simulink model "model"  (R2014a)
(part 2 of 3)

  _CN_86577898_150000_CN_136543640_150000 : powerlib/Elements/Distributed Parameters Line  Phases=3  Frequency=60  Resistance=[0.01273 0.3864]  Inductance="[0.9337e-3  4.1264e-3]"  Capacitance=[12.74e-9 7.751e-9]  Length=52.261  x1=[0 0 0 0; 0.0001244 0 0 0; 0.0002488 0 0 0; 0.0003733 0 0 0; 0.0004977 0 0 0; 0.0006221 0 0 0]  x2=[0 0 0 0; 0.0001244 0 0 0; 0.0002488 0 0 0; 0.0003733 0 0 0; 0.0004977 0 0 0; 0.0006221 0 0 0]  x3=[0 0 0 0; 0.0001244 0 0 0; 0.0002488 0 0 0; 0.0003733 0 0 0; 0.0004977 0 0 0; 0.0006221 0 0 0]  x4=[0 0 0 0; 0.0001244 0 0 0; 0.0002488 0 0 0; 0.0003733 0 0 0; 0.0004977 0 0 0; 0.0006221 0 0 0]  x5=0  V1=ones(3,3)  V2=ones(3,3)  I1=ones(3,3)  I2=ones(3,3)  nHarmo=1  Measurements=None
  _CN_92352843_150000_CN_149922043_150000 : powerlib/Elements/Distributed Parameters Line  Phases=3  Frequency=60  Resistance=[0.01273 0.3864]  Inductance="[0.9337e-3  4.1264e-3]"  Capacitance=[12.74e-9 7.751e-9]  Length=68.3675  x1=[0 0 0 0; 0.0001244 0 0 0; 0.0002488 0 0 0; 0.0003733 0 0 0; 0.0004977 0 0 0; 0.0006221 0 0 0]  x2=[0 0 0 0; 0.0001244 0 0 0; 0.0002488 0 0 0; 0.0003733 0 0 0; 0.0004977 0 0 0; 0.0006221 0 0 0]  x3=[0 0 0 0; 0.0001244 0 0 0; 0.0002488 0 0 0; 0.0003733 0 0 0; 0.0004977 0 0 0; 0.0006221 0 0 0]  x4=[0 0 0 0; 0.0001244 0 0 0; 0.0002488 0 0 0; 0.0003733 0 0 0; 0.0004977 0 0 0; 0.0006221 0 0 0]  x5=0  V1=ones(3,3)  V2=ones(3,3)  I1=ones(3,3)  I2=ones(3,3)  nHarmo=1  Measurements=None
  _CN_92611147_150000_CN_85646787_150000 : powerlib/Elements/Distributed Parameters Line  Phases=3  Frequency=60  Resistance=[0.01273 0.3864]  Inductance="[0.9337e-3  4.1264e-3]"  Capacitance=[12.74e-9 7.751e-9]  Length=4.1516  x1=[0 0 0 0; 0.0001244 0 0 0; 0.0002488 0 0 0; 0.0003733 0 0 0; 0.0004977 0 0 0; 0.0006221 0 0 0]  x2=[0 0 0 0; 0.0001244 0 0 0; 0.0002488 0 0 0; 0.0003733 0 0 0; 0.0004977 0 0 0; 0.0006221 0 0 0]  x3=[0 0 0 0; 0.0001244 0 0 0; 0.0002488 0 0 0; 0.0003733 0 0 0; 0.0004977 0 0 0; 0.0006221 0 0 0]  x4=[0 0 0 0; 0.0001244 0 0 0; 0.0002488 0 0 0; 0.0003733 0 0 0; 0.0004977 0 0 0; 0.0006221 0 0 0]  x5=0  V1=ones(3,3)  V2=ones(3,3)  I1=ones(3,3)  I2=ones(3,3)  nHarmo=1  Measurements=None
  _CN_92611161_150000_CN_85646787_150000 : powerlib/Elements/Distributed Parameters Line  Phases=3  Frequency=60  Resistance=[0.01273 0.3864]  Inductance="[0.9337e-3  4.1264e-3]"  Capacitance=[12.74e-9 7.751e-9]  Length=18.2958  x1=[0 0 0 0; 0.0001244 0 0 0; 0.0002488 0 0 0; 0.0003733 0 0 0; 0.0004977 0 0 0; 0.0006221 0 0 0]  x2=[0 0 0 0; 0.0001244 0 0 0; 0.0002488 0 0 0; 0.0003733 0 0 0; 0.0004977 0 0 0; 0.0006221 0 0 0]  x3=[0 0 0 0; 0.0001244 0 0 0; 0.0002488 0 0 0; 0.0003733 0 0 0; 0.0004977 0 0 0; 0.0006221 0 0 0]  x4=[0 0 0 0; 0.0001244 0 0 0; 0.0002488 0 0 0; 0.0003733 0 0 0; 0.0004977 0 0 0; 0.0006221 0 0 0]  x5=0  V1=ones(3,3)  V2=ones(3,3)  I1=ones(3,3)  I2=ones(3,3)  nHarmo=1  Measurements=None
  _CN_92611161_150000_CN_92611154_150000 : powerlib/Elements/Distributed Parameters Line  Phases=3  Frequency=60  Resistance=[0.01273 0.3864]  Inductance="[0.9337e-3  4.1264e-3]"  Capacitance=[12.74e-9 7.751e-9]  Length=4.6182  x1=[0 0 0 0; 0.0001244 0 0 0; 0.0002488 0 0 0; 0.0003733 0 0 0; 0.0004977 0 0 0; 0.0006221 0 0 0]  x2=[0 0 0 0; 0.0001244 0 0 0; 0.0002488 0 0 0; 0.0003733 0 0 0; 0.0004977 0 0 0; 0.0006221 0 0 0]  x3=[0 0 0 0; 0.0001244 0 0 0; 0.0002488 0 0 0; 0.0003733 0 0 0; 0.0004977 0 0 0; 0.0006221 0 0 0]  x4=[0 0 0 0; 0.0001244 0 0 0; 0.0002488 0 0 0; 0.0003733 0 0 0; 0.0004977 0 0 0; 0.0006221 0 0 0]  x5=0  V1=ones(3,3)  V2=ones(3,3)  I1=ones(3,3)  I2=ones(3,3)  nHarmo=1  Measurements=None
  _CN_93061385_150000_CN_93061390_150000 : powerlib/Elements/Distributed Parameters Line  Phases=3  Frequency=60  Resistance=[0.01273 0.3864]  Inductance="[0.9337e-3  4.1264e-3]"  Capacitance=[12.74e-9 7.751e-9]  Length=5.508  x1=[0 0 0 0; 0.0001244 0 0 0; 0.0002488 0 0 0; 0.0003733 0 0 0; 0.0004977 0 0 0; 0.0006221 0 0 0]  x2=[0 0 0 0; 0.0001244 0 0 0; 0.0002488 0 0 0; 0.0003733 0 0 0; 0.0004977 0 0 0; 0.0006221 0 0 0]  x3=[0 0 0 0; 0.0001244 0 0 0; 0.0002488 0 0 0; 0.0003733 0 0 0; 0.0004977 0 0 0; 0.0006221 0 0 0]  x4=[0 0 0 0; 0.0001244 0 0 0; 0.0002488 0 0 0; 0.0003733 0 0 0; 0.0004977 0 0 0; 0.0006221 0 0 0]  x5=0  V1=ones(3,3)  V2=ones(3,3)  I1=ones(3,3)  I2=ones(3,3)  nHarmo=1  Measurements=None
  _CN_93061390_150000_CN_115027244_150000 : powerlib/Elements/Distributed Parameters Line  Phases=3  Frequency=60  Resistance=[0.01273 0.3864]  Inductance="[0.9337e-3  4.1264e-3]"  Capacitance=[12.74e-9 7.751e-9]  Length=7.1152  x1=[0 0 0 0; 0.0001244 0 0 0; 0.0002488 0 0 0; 0.0003733 0 0 0; 0.0004977 0 0 0; 0.0006221 0 0 0]  x2=[0 0 0 0; 0.0001244 0 0 0; 0.0002488 0 0 0; 0.0003733 0 0 0; 0.0004977 0 0 0; 0.0006221 0 0 0]  x3=[0 0 0 0; 0.0001244 0 0 0; 0.0002488 0 0 0; 0.0003733 0 0 0; 0.0004977 0 0 0; 0.0006221 0 0 0]  x4=[0 0 0 0; 0.0001244 0 0 0; 0.0002488 0 0 0; 0.0003733 0 0 0; 0.0004977 0 0 0; 0.0006221 0 0 0]  x5=0  V1=ones(3,3)  V2=ones(3,3)  I1=ones(3,3)  I2=ones(3,3)  nHarmo=1  Measurements=None
  _CN_93085785_150000_CN_93085804_150000 : powerlib/Elements/Distributed Parameters Line  Phases=3  Frequency=60  Resistance=[0.01273 0.3864]  Inductance="[0.9337e-3  4.1264e-3]"  Capacitance=[12.74e-9 7.751e-9]  Length=0.70246  x1=[0 0 0 0; 0.0001244 0 0 0; 0.0002488 0 0 0; 0.0003733 0 0 0; 0.0004977 0 0 0; 0.0006221 0 0 0]  x2=[0 0 0 0; 0.0001244 0 0 0; 0.0002488 0 0 0; 0.0003733 0 0 0; 0.0004977 0 0 0; 0.0006221 0 0 0]  x3=[0 0 0 0; 0.0001244 0 0 0; 0.0002488 0 0 0; 0.0003733 0 0 0; 0.0004977 0 0 0; 0.0006221 0 0 0]  x4=[0 0 0 0; 0.0001244 0 0 0; 0.0002488 0 0 0; 0.0003733 0 0 0; 0.0004977 0 0 0; 0.0006221 0 0 0]  x5=0  V1=ones(3,3)  V2=ones(3,3)  I1=ones(3,3)  I2=ones(3,3)  nHarmo=1  Measurements=None
  _CN_93085804_150000_CN_93061390_150000 : powerlib/Elements/Distributed Parameters Line  Phases=3  Frequency=60  Resistance=[0.01273 0.3864]  Inductance="[0.9337e-3  4.1264e-3]"  Capacitance=[12.74e-9 7.751e-9]  Length=9.0251  x1=[0 0 0 0; 0.0001244 0 0 0; 0.0002488 0 0 0; 0.0003733 0 0 0; 0.0004977 0 0 0; 0.0006221 0 0 0]  x2=[0 0 0 0; 0.0001244 0 0 0; 0.0002488 0 0 0; 0.0003733 0 0 0; 0.0004977 0 0 0; 0.0006221 0 0 0]  x3=[0 0 0 0; 0.0001244 0 0 0; 0.0002488 0 0 0; 0.0003733 0 0 0; 0.0004977 0 0 0; 0.0006221 0 0 0]  x4=[0 0 0 0; 0.0001244 0 0 0; 0.0002488 0 0 0; 0.0003733 0 0 0; 0.0004977 0 0 0; 0.0006221 0 0 0]  x5=0  V1=ones(3,3)  V2=ones(3,3)  I1=ones(3,3)  I2=ones(3,3)  nHarmo=1  Measurements=None
  _CN_93119207_400000_CN_86577898_400000 : powerlib/Elements/Distributed Parameters Line  Phases=3  Frequency=60  Resistance=[0.01273 0.3864]  Inductance="[0.9337e-3  4.1264e-3]"  Capacitance=[12.74e-9 7.751e-9]  Length=76.386  x1=[0 0 0 0; 0.0001244 0 0 0; 0.0002488 0 0 0; 0.0003733 0 0 0; 0.0004977 0 0 0; 0.0006221 0 0 0]  x2=[0 0 0 0; 0.0001244 0 0 0; 0.0002488 0 0 0; 0.0003733 0 0 0; 0.0004977 0 0 0; 0.0006221 0 0 0]  x3=[0 0 0 0; 0.0001244 0 0 0; 0.0002488 0 0 0; 0.0003733 0 0 0; 0.0004977 0 0 0; 0.0006221 0 0 0]  x4=[0 0 0 0; 0.0001244 0 0 0; 0.0002488 0 0 0; 0.0003733 0 0 0; 0.0004977 0 0 0; 0.0006221 0 0 0]  x5=0  V1=ones(3,3)  V2=ones(3,3)  I1=ones(3,3)  I2=ones(3,3)  nHarmo=1  Measurements=None
  _CN_93173562_150000_CN_93172457_150000 : powerlib/Elements/Distributed Parameters Line  Phases=3  Frequency=60  Resistance=[0.01273 0.3864]  Inductance="[0.9337e-3  4.1264e-3]"  Capacitance=[12.74e-9 7.751e-9]  Length=18.3315  x1=[0 0 0 0; 0.0001244 0 0 0; 0.0002488 0 0 0; 0.0003733 0 0 0; 0.0004977 0 0 0; 0.0006221 0 0 0]  x2=[0 0 0 0; 0.0001244 0 0 0; 0.0002488 0 0 0; 0.0003733 0 0 0; 0.0004977 0 0 0; 0.0006221 0 0 0]  x3=[0 0 0 0; 0.0001244 0 0 0; 0.0002488 0 0 0; 0.0003733 0 0 0; 0.0004977 0 0 0; 0.0006221 0 0 0]  x4=[0 0 0 0; 0.0001244 0 0 0; 0.0002488 0 0 0; 0.0003733 0 0 0; 0.0004977 0 0 0; 0.0006221 0 0 0]  x5=0  V1=ones(3,3)  V2=ones(3,3)  I1=ones(3,3)  I2=ones(3,3)  nHarmo=1  Measurements=None
  _CN_93383685_150000_CN_135706289_150000 : powerlib/Elements/Distributed Parameters Line  Phases=3  Frequency=60  Resistance=[0.01273 0.3864]  Inductance="[0.9337e-3  4.1264e-3]"  Capacitance=[12.74e-9 7.751e-9]  Length=36.1686  x1=[0 0 0 0; 0.0001244 0 0 0; 0.0002488 0 0 0; 0.0003733 0 0 0; 0.0004977 0 0 0; 0.0006221 0 0 0]  x2=[0 0 0 0; 0.0001244 0 0 0; 0.0002488 0 0 0; 0.0003733 0 0 0; 0.0004977 0 0 0; 0.0006221 0 0 0]  x3=[0 0 0 0; 0.0001244 0 0 0; 0.0002488 0 0 0; 0.0003733 0 0 0; 0.0004977 0 0 0; 0.0006221 0 0 0]  x4=[0 0 0 0; 0.0001244 0 0 0; 0.0002488 0 0 0; 0.0003733 0 0 0; 0.0004977 0 0 0; 0.0006221 0 0 0]  x5=0  V1=ones(3,3)  V2=ones(3,3)  I1=ones(3,3)  I2=ones(3,3)  nHarmo=1  Measurements=None
  _CN_93383685_150000_CN_15642023_150000 : powerlib/Elements/Distributed Parameters Line  Phases=3  Frequency=60  Resistance=[0.01273 0.3864]  Inductance="[0.9337e-3  4.1264e-3]"  Capacitance=[12.74e-9 7.751e-9]  Length=0.77584  x1=[0 0 0 0; 0.0001244 0 0 0; 0.0002488 0 0 0; 0.0003733 0 0 0; 0.0004977 0 0 0; 0.0006221 0 0 0]  x2=[0 0 0 0; 0.0001244 0 0 0; 0.0002488 0 0 0; 0.0003733 0 0 0; 0.0004977 0 0 0; 0.0006221 0 0 0]  x3=[0 0 0 0; 0.0001244 0 0 0; 0.0002488 0 0 0; 0.0003733 0 0 0; 0.0004977 0 0 0; 0.0006221 0 0 0]  x4=[0 0 0 0; 0.0001244 0 0 0; 0.0002488 0 0 0; 0.0003733 0 0 0; 0.0004977 0 0 0; 0.0006221 0 0 0]  x5=0  V1=ones(3,3)  V2=ones(3,3)  I1=ones(3,3)  I2=ones(3,3)  nHarmo=1  Measurements=None
  _CN_93383685_400000_CN_149672244_400000 : powerlib/Elements/Distributed Parameters Line  Phases=3  Frequency=60  Resistance=[0.01273 0.3864]  Inductance="[0.9337e-3  4.1264e-3]"  Capacitance=[12.74e-9 7.751e-9]  Length=35.3897  x1=[0 0 0 0; 0.0001244 0 0 0; 0.0002488 0 0 0; 0.0003733 0 0 0; 0.0004977 0 0 0; 0.0006221 0 0 0]  x2=[0 0 0 0; 0.0001244 0 0 0; 0.0002488 0 0 0; 0.0003733 0 0 0; 0.0004977 0 0 0; 0.0006221 0 0 0]  x3=[0 0 0 0; 0.0001244 0 0 0; 0.0002488 0 0 0; 0.0003733 0 0 0; 0.0004977 0 0 0; 0.0006221 0 0 0]  x4=[0 0 0 0; 0.0001244 0 0 0; 0.0002488 0 0 0; 0.0003733 0 0 0; 0.0004977 0 0 0; 0.0006221 0 0 0]  x5=0  V1=ones(3,3)  V2=ones(3,3)  I1=ones(3,3)  I2=ones(3,3)  nHarmo=1  Measurements=None
  _CN_93383685_400000_CN_15641949_400000 : powerlib/Elements/Distributed Parameters Line  Phases=3  Frequency=60  Resistance=[0.01273 0.3864]  Inductance="[0.9337e-3  4.1264e-3]"  Capacitance=[12.74e-9 7.751e-9]  Length=15.3876  x1=[0 0 0 0; 0.0001244 0 0 0; 0.0002488 0 0 0; 0.0003733 0 0 0; 0.0004977 0 0 0; 0.0006221 0 0 0]  x2=[0 0 0 0; 0.0001244 0 0 0; 0.0002488 0 0 0; 0.0003733 0 0 0; 0.0004977 0 0 0; 0.0006221 0 0 0]  x3=[0 0 0 0; 0.0001244 0 0 0; 0.0002488 0 0 0; 0.0003733 0 0 0; 0.0004977 0 0 0; 0.0006221 0 0 0]  x4=[0 0 0 0; 0.0001244 0 0 0; 0.0002488 0 0 0; 0.0003733 0 0 0; 0.0004977 0 0 0; 0.0006221 0 0 0]  x5=0  V1=ones(3,3)  V2=ones(3,3)  I1=ones(3,3)  I2=ones(3,3)  nHarmo=1  Measurements=None
  _CN_93383685_400000_CN_15642023_150000 : powerlib/Elements/Distributed Parameters Line  Phases=3  Frequency=60  Resistance=[0.01273 0.3864]  Inductance="[0.9337e-3  4.1264e-3]"  Capacitance=[12.74e-9 7.751e-9]  Length=0.4473  x1=[0 0 0 0; 0.0001244 0 0 0; 0.0002488 0 0 0; 0.0003733 0 0 0; 0.0004977 0 0 0; 0.0006221 0 0 0]  x2=[0 0 0 0; 0.0001244 0 0 0; 0.0002488 0 0 0; 0.0003733 0 0 0; 0.0004977 0 0 0; 0.0006221 0 0 0]  x3=[0 0 0 0; 0.0001244 0 0 0; 0.0002488 0 0 0; 0.0003733 0 0 0; 0.0004977 0 0 0; 0.0006221 0 0 0]  x4=[0 0 0 0; 0.0001244 0 0 0; 0.0002488 0 0 0; 0.0003733 0 0 0; 0.0004977 0 0 0; 0.0006221 0 0 0]  x5=0  V1=ones(3,3)  V2=ones(3,3)  I1=ones(3,3)  I2=ones(3,3)  nHarmo=1  Measurements=None
  _CN_93383685_400000_CN_171506480_400000 : powerlib/Elements/Distributed Parameters Line  Phases=3  Frequency=60  Resistance=[0.01273 0.3864]  Inductance="[0.9337e-3  4.1264e-3]"  Capacitance=[12.74e-9 7.751e-9]  Length=49.411  x1=[0 0 0 0; 0.0001244 0 0 0; 0.0002488 0 0 0; 0.0003733 0 0 0; 0.0004977 0 0 0; 0.0006221 0 0 0]  x2=[0 0 0 0; 0.0001244 0 0 0; 0.0002488 0 0 0; 0.0003733 0 0 0; 0.0004977 0 0 0; 0.0006221 0 0 0]  x3=[0 0 0 0; 0.0001244 0 0 0; 0.0002488 0 0 0; 0.0003733 0 0 0; 0.0004977 0 0 0; 0.0006221 0 0 0]  x4=[0 0 0 0; 0.0001244 0 0 0; 0.0002488 0 0 0; 0.0003733 0 0 0; 0.0004977 0 0 0; 0.0006221 0 0 0]  x5=0  V1=ones(3,3)  V2=ones(3,3)  I1=ones(3,3)  I2=ones(3,3)  nHarmo=1  Measurements=None
  _CN_93383685_400000_CN_249066440_400000 : powerlib/Elements/Distributed Parameters Line  Phases=3  Frequency=60  Resistance=[0.01273 0.3864]  Inductance="[0.9337e-3  4.1264e-3]"  Capacitance=[12.74e-9 7.751e-9]  Length=18.7994  x1=[0 0 0 0; 0.0001244 0 0 0; 0.0002488 0 0 0; 0.0003733 0 0 0; 0.0004977 0 0 0; 0.0006221 0 0 0]  x2=[0 0 0 0; 0.0001244 0 0 0; 0.0002488 0 0 0; 0.0003733 0 0 0; 0.0004977 0 0 0; 0.0006221 0 0 0]  x3=[0 0 0 0; 0.0001244 0 0 0; 0.0002488 0 0 0; 0.0003733 0 0 0; 0.0004977 0 0 0; 0.0006221 0 0 0]  x4=[0 0 0 0; 0.0001244 0 0 0; 0.0002488 0 0 0; 0.0003733 0 0 0; 0.0004977 0 0 0; 0.0006221 0 0 0]  x5=0  V1=ones(3,3)  V2=ones(3,3)  I1=ones(3,3)  I2=ones(3,3)  nHarmo=1  Measurements=None
  _CN_93383685_400000_CN_86577898_400000 : powerlib/Elements/Distributed Parameters Line  Phases=3  Frequency=60  Resistance=[0.01273 0.3864]  Inductance="[0.9337e-3  4.1264e-3]"  Capacitance=[12.74e-9 7.751e-9]  Length=53.9293  x1=[0 0 0 0; 0.0001244 0 0 0; 0.0002488 0 0 0; 0.0003733 0 0 0; 0.0004977 0 0 0; 0.0006221 0 0 0]  x2=[0 0 0 0; 0.0001244 0 0 0; 0.0002488 0 0 0; 0.0003733 0 0 0; 0.0004977 0 0 0; 0.0006221 0 0 0]  x3=[0 0 0 0; 0.0001244 0 0 0; 0.0002488 0 0 0; 0.0003733 0 0 0; 0.0004977 0 0 0; 0.0006221 0 0 0]  x4=[0 0 0 0; 0.0001244 0 0 0; 0.0002488 0 0 0; 0.0003733 0 0 0; 0.0004977 0 0 0; 0.0006221 0 0 0]  x5=0  V1=ones(3,3)  V2=ones(3,3)  I1=ones(3,3)  I2=ones(3,3)  nHarmo=1  Measurements=None
  _CN_93906290_150000_CN_93906327_150000 : powerlib/Elements/Distributed Parameters Line  Phases=3  Frequency=60  Resistance=[0.01273 0.3864]  Inductance="[0.9337e-3  4.1264e-3]"  Capacitance=[12.74e-9 7.751e-9]  Length=20.4524  x1=[0 0 0 0; 0.0001244 0 0 0; 0.0002488 0 0 0; 0.0003733 0 0 0; 0.0004977 0 0 0; 0.0006221 0 0 0]  x2=[0 0 0 0; 0.0001244 0 0 0; 0.0002488 0 0 0; 0.0003733 0 0 0; 0.0004977 0 0 0; 0.0006221 0 0 0]  x3=[0 0 0 0; 0.0001244 0 0 0; 0.0002488 0 0 0; 0.0003733 0 0 0; 0.0004977 0 0 0; 0.0006221 0 0 0]  x4=[0 0 0 0; 0.0001244 0 0 0; 0.0002488 0 0 0; 0.0003733 0 0 0; 0.0004977 0 0 0; 0.0006221 0 0 0]  x5=0  V1=ones(3,3)  V2=ones(3,3)  I1=ones(3,3)  I2=ones(3,3)  nHarmo=1  Measurements=None
  _CN_95989793_150000_CN_92352843_150000 : powerlib/Elements/Distributed Parameters Line  Phases=3  Frequency=60  Resistance=[0.01273 0.3864]  Inductance="[0.9337e-3  4.1264e-3]"  Capacitance=[12.74e-9 7.751e-9]  Length=5.9887  x1=[0 0 0 0; 0.0001244 0 0 0; 0.0002488 0 0 0; 0.0003733 0 0 0; 0.0004977 0 0 0; 0.0006221 0 0 0]  x2=[0 0 0 0; 0.0001244 0 0 0; 0.0002488 0 0 0; 0.0003733 0 0 0; 0.0004977 0 0 0; 0.0006221 0 0 0]  x3=[0 0 0 0; 0.0001244 0 0 0; 0.0002488 0 0 0; 0.0003733 0 0 0; 0.0004977 0 0 0; 0.0006221 0 0 0]  x4=[0 0 0 0; 0.0001244 0 0 0; 0.0002488 0 0 0; 0.0003733 0 0 0; 0.0004977 0 0 0; 0.0006221 0 0 0]  x5=0  V1=ones(3,3)  V2=ones(3,3)  I1=ones(3,3)  I2=ones(3,3)  nHarmo=1  Measurements=None
  _CN_96020492_150000_CN_96314289_150000 : powerlib/Elements/Distributed Parameters Line  Phases=3  Frequency=60  Resistance=[0.01273 0.3864]  Inductance="[0.9337e-3  4.1264e-3]"  Capacitance=[12.74e-9 7.751e-9]  Length=14.9727  x1=[0 0 0 0; 0.0001244 0 0 0; 0.0002488 0 0 0; 0.0003733 0 0 0; 0.0004977 0 0 0; 0.0006221 0 0 0]  x2=[0 0 0 0; 0.0001244 0 0 0; 0.0002488 0 0 0; 0.0003733 0 0 0; 0.0004977 0 0 0; 0.0006221 0 0 0]  x3=[0 0 0 0; 0.0001244 0 0 0; 0.0002488 0 0 0; 0.0003733 0 0 0; 0.0004977 0 0 0; 0.0006221 0 0 0]  x4=[0 0 0 0; 0.0001244 0 0 0; 0.0002488 0 0 0; 0.0003733 0 0 0; 0.0004977 0 0 0; 0.0006221 0 0 0]  x5=0  V1=ones(3,3)  V2=ones(3,3)  I1=ones(3,3)  I2=ones(3,3)  nHarmo=1  Measurements=None
  _CN_96040696_150000_CN_96040682_150000 : powerlib/Elements/Distributed Parameters Line  Phases=3  Frequency=60  Resistance=[0.01273 0.3864]  Inductance="[0.9337e-3  4.1264e-3]"  Capacitance=[12.74e-9 7.751e-9]  Length=5.757  x1=[0 0 0 0; 0.0001244 0 0 0; 0.0002488 0 0 0; 0.0003733 0 0 0; 0.0004977 0 0 0; 0.0006221 0 0 0]  x2=[0 0 0 0; 0.0001244 0 0 0; 0.0002488 0 0 0; 0.0003733 0 0 0; 0.0004977 0 0 0; 0.0006221 0 0 0]  x3=[0 0 0 0; 0.0001244 0 0 0; 0.0002488 0 0 0; 0.0003733 0 0 0; 0.0004977 0 0 0; 0.0006221 0 0 0]  x4=[0 0 0 0; 0.0001244 0 0 0; 0.0002488 0 0 0; 0.0003733 0 0 0; 0.0004977 0 0 0; 0.0006221 0 0 0]  x5=0  V1=ones(3,3)  V2=ones(3,3)  I1=ones(3,3)  I2=ones(3,3)  nHarmo=1  Measurements=None
  _CN_96040696_150000_CN_96314284_150000 : powerlib/Elements/Distributed Parameters Line  Phases=3  Frequency=60  Resistance=[0.01273 0.3864]  Inductance="[0.9337e-3  4.1264e-3]"  Capacitance=[12.74e-9 7.751e-9]  Length=6.6971  x1=[0 0 0 0; 0.0001244 0 0 0; 0.0002488 0 0 0; 0.0003733 0 0 0; 0.0004977 0 0 0; 0.0006221 0 0 0]  x2=[0 0 0 0; 0.0001244 0 0 0; 0.0002488 0 0 0; 0.0003733 0 0 0; 0.0004977 0 0 0; 0.0006221 0 0 0]  x3=[0 0 0 0; 0.0001244 0 0 0; 0.0002488 0 0 0; 0.0003733 0 0 0; 0.0004977 0 0 0; 0.0006221 0 0 0]  x4=[0 0 0 0; 0.0001244 0 0 0; 0.0002488 0 0 0; 0.0003733 0 0 0; 0.0004977 0 0 0; 0.0006221 0 0 0]  x5=0  V1=ones(3,3)  V2=ones(3,3)  I1=ones(3,3)  I2=ones(3,3)  nHarmo=1  Measurements=None
  _CN_96040696_150000_CN_96314286_150000 : powerlib/Elements/Distributed Parameters Line  Phases=3  Frequency=60  Resistance=[0.01273 0.3864]  Inductance="[0.9337e-3  4.1264e-3]"  Capacitance=[12.74e-9 7.751e-9]  Length=13.1913  x1=[0 0 0 0; 0.0001244 0 0 0; 0.0002488 0 0 0; 0.0003733 0 0 0; 0.0004977 0 0 0; 0.0006221 0 0 0]  x2=[0 0 0 0; 0.0001244 0 0 0; 0.0002488 0 0 0; 0.0003733 0 0 0; 0.0004977 0 0 0; 0.0006221 0 0 0]  x3=[0 0 0 0; 0.0001244 0 0 0; 0.0002488 0 0 0; 0.0003733 0 0 0; 0.0004977 0 0 0; 0.0006221 0 0 0]  x4=[0 0 0 0; 0.0001244 0 0 0; 0.0002488 0 0 0; 0.0003733 0 0 0; 0.0004977 0 0 0; 0.0006221 0 0 0]  x5=0  V1=ones(3,3)  V2=ones(3,3)  I1=ones(3,3)  I2=ones(3,3)  nHarmo=1  Measurements=None
  _CN_96040696_150000_CN_96314289_150000 : powerlib/Elements/Distributed Parameters Line  Phases=3  Frequency=60  Resistance=[0.01273 0.3864]  Inductance="[0.9337e-3  4.1264e-3]"  Capacitance=[12.74e-9 7.751e-9]  Length=7.9542  x1=[0 0 0 0; 0.0001244 0 0 0; 0.0002488 0 0 0; 0.0003733 0 0 0; 0.0004977 0 0 0; 0.0006221 0 0 0]  x2=[0 0 0 0; 0.0001244 0 0 0; 0.0002488 0 0 0; 0.0003733 0 0 0; 0.0004977 0 0 0; 0.0006221 0 0 0]  x3=[0 0 0 0; 0.0001244 0 0 0; 0.0002488 0 0 0; 0.0003733 0 0 0; 0.0004977 0 0 0; 0.0006221 0 0 0]  x4=[0 0 0 0; 0.0001244 0 0 0; 0.0002488 0 0 0; 0.0003733 0 0 0; 0.0004977 0 0 0; 0.0006221 0 0 0]  x5=0  V1=ones(3,3)  V2=ones(3,3)  I1=ones(3,3)  I2=ones(3,3)  nHarmo=1  Measurements=None
  _CN_96314286_150000_CN_96314289_150000 : powerlib/Elements/Distributed Parameters Line  Phases=3  Frequency=60  Resistance=[0.01273 0.3864]  Inductance="[0.9337e-3  4.1264e-3]"  Capacitance=[12.74e-9 7.751e-9]  Length=3.0156  x1=[0 0 0 0; 0.0001244 0 0 0; 0.0002488 0 0 0; 0.0003733 0 0 0; 0.0004977 0 0 0; 0.0006221 0 0 0]  x2=[0 0 0 0; 0.0001244 0 0 0; 0.0002488 0 0 0; 0.0003733 0 0 0; 0.0004977 0 0 0; 0.0006221 0 0 0]  x3=[0 0 0 0; 0.0001244 0 0 0; 0.0002488 0 0 0; 0.0003733 0 0 0; 0.0004977 0 0 0; 0.0006221 0 0 0]  x4=[0 0 0 0; 0.0001244 0 0 0; 0.0002488 0 0 0; 0.0003733 0 0 0; 0.0004977 0 0 0; 0.0006221 0 0 0]  x5=0  V1=ones(3,3)  V2=ones(3,3)  I1=ones(3,3)  I2=ones(3,3)  nHarmo=1  Measurements=None
  _CN_96759614_150000_CN_128799211_150000 : powerlib/Elements/Distributed Parameters Line  Phases=3  Frequency=60  Resistance=[0.01273 0.3864]  Inductance="[0.9337e-3  4.1264e-3]"  Capacitance=[12.74e-9 7.751e-9]  Length=41.7594  x1=[0 0 0 0; 0.0001244 0 0 0; 0.0002488 0 0 0; 0.0003733 0 0 0; 0.0004977 0 0 0; 0.0006221 0 0 0]  x2=[0 0 0 0; 0.0001244 0 0 0; 0.0002488 0 0 0; 0.0003733 0 0 0; 0.0004977 0 0 0; 0.0006221 0 0 0]  x3=[0 0 0 0; 0.0001244 0 0 0; 0.0002488 0 0 0; 0.0003733 0 0 0; 0.0004977 0 0 0; 0.0006221 0 0 0]  x4=[0 0 0 0; 0.0001244 0 0 0; 0.0002488 0 0 0; 0.0003733 0 0 0; 0.0004977 0 0 0; 0.0006221 0 0 0]  x5=0  V1=ones(3,3)  V2=ones(3,3)  I1=ones(3,3)  I2=ones(3,3)  nHarmo=1  Measurements=None
  bus1 : powerlib/Measurements/Load Flow Bus  LConnTagsString=a  ID=bus1  Vbase=150000  Vref=1  Vangle=0  VLF=1  angleLF=0
      settings: AttributesFormatString=|
      | %<ID>
      | %<Vbase>V
      | %<VLF>pu
      | %<angleLF>deg.
      | %<Name>
  bus10 : powerlib/Measurements/Load Flow Bus  LConnTagsString=a  ID=bus10  Vbase=150000  Vref=1  Vangle=0  VLF=1  angleLF=0
      settings: AttributesFormatString=|
      | %<ID>
      | %<Vbase>V
      | %<VLF>pu
      | %<angleLF>deg.
      | %<Name>
  bus100 : powerlib/Measurements/Load Flow Bus  LConnTagsString=a  ID=bus100  Vbase=150000  Vref=1  Vangle=0  VLF=1  angleLF=0
      settings: AttributesFormatString=|
      | %<ID>
      | %<Vbase>V
      | %<VLF>pu
      | %<angleLF>deg.
      | %<Name>
  bus101 : powerlib/Measurements/Load Flow Bus  LConnTagsString=a  ID=bus101  Vbase=150000  Vref=1  Vangle=0  VLF=1  angleLF=0
      settings: AttributesFormatString=|
      | %<ID>
      | %<Vbase>V
      | %<VLF>pu
      | %<angleLF>deg.
      | %<Name>
  bus102 : powerlib/Measurements/Load Flow Bus  LConnTagsString=a  ID=bus102  Vbase=150000  Vref=1  Vangle=0  VLF=1  angleLF=0
      settings: AttributesFormatString=|
      | %<ID>
      | %<Vbase>V
      | %<VLF>pu
      | %<angleLF>deg.
      | %<Name>
  bus103 : powerlib/Measurements/Load Flow Bus  LConnTagsString=a  ID=bus103  Vbase=150000  Vref=1  Vangle=0  VLF=1  angleLF=0
      settings: AttributesFormatString=|
      | %<ID>
      | %<Vbase>V
      | %<VLF>pu
      | %<angleLF>deg.
      | %<Name>
  bus104 : powerlib/Measurements/Load Flow Bus  LConnTagsString=a  ID=bus104  Vbase=150000  Vref=1  Vangle=0  VLF=1  angleLF=0
      settings: AttributesFormatString=|
      | %<ID>
      | %<Vbase>V
      | %<VLF>pu
      | %<angleLF>deg.
      | %<Name>
  bus105 : powerlib/Measurements/Load Flow Bus  LConnTagsString=a  ID=bus105  Vbase=150000  Vref=1  Vangle=0  VLF=1  angleLF=0
      settings: AttributesFormatString=|
      | %<ID>
      | %<Vbase>V
      | %<VLF>pu
      | %<angleLF>deg.
      | %<Name>
  bus106 : powerlib/Measurements/Load Flow Bus  LConnTagsString=a  ID=bus106  Vbase=150000  Vref=1  Vangle=0  VLF=1  angleLF=0
      settings: AttributesFormatString=|
      | %<ID>
      | %<Vbase>V
      | %<VLF>pu
      | %<angleLF>deg.
      | %<Name>
  bus107 : powerlib/Measurements/Load Flow Bus  LConnTagsString=a  ID=bus107  Vbase=150000  Vref=1  Vangle=0  VLF=1  angleLF=0
      settings: AttributesFormatString=|
      | %<ID>
      | %<Vbase>V
      | %<VLF>pu
      | %<angleLF>deg.
      | %<Name>
  bus108 : powerlib/Measurements/Load Flow Bus  LConnTagsString=a  ID=bus108  Vbase=150000  Vref=1  Vangle=0  VLF=1  angleLF=0
      settings: AttributesFormatString=|
      | %<ID>
      | %<Vbase>V
      | %<VLF>pu
      | %<angleLF>deg.
      | %<Name>
  bus109 : powerlib/Measurements/Load Flow Bus  LConnTagsString=a  ID=bus109  Vbase=150000  Vref=1  Vangle=0  VLF=1  angleLF=0
      settings: AttributesFormatString=|
      | %<ID>
      | %<Vbase>V
      | %<VLF>pu
      | %<angleLF>deg.
      | %<Name>
  bus11 : powerlib/Measurements/Load Flow Bus  LConnTagsString=a  ID=bus11  Vbase=150000  Vref=1  Vangle=0  VLF=1  angleLF=0
      settings: AttributesFormatString=|
      | %<ID>
      | %<Vbase>V
      | %<VLF>pu
      | %<angleLF>deg.
      | %<Name>
  bus110 : powerlib/Measurements/Load Flow Bus  LConnTagsString=a  ID=bus110  Vbase=150000  Vref=1  Vangle=0  VLF=1  angleLF=0
      settings: AttributesFormatString=|
      | %<ID>
      | %<Vbase>V
      | %<VLF>pu
      | %<angleLF>deg.
      | %<Name>
  bus111 : powerlib/Measurements/Load Flow Bus  LConnTagsString=a  ID=bus111  Vbase=150000  Vref=1  Vangle=0  VLF=1  angleLF=0
      settings: AttributesFormatString=|
      | %<ID>
      | %<Vbase>V
      | %<VLF>pu
      | %<angleLF>deg.
      | %<Name>
  bus112 : powerlib/Measurements/Load Flow Bus  LConnTagsString=a  ID=bus112  Vbase=150000  Vref=1  Vangle=0  VLF=1  angleLF=0
      settings: AttributesFormatString=|
      | %<ID>
      | %<Vbase>V
      | %<VLF>pu
      | %<angleLF>deg.
      | %<Name>
  bus113 : powerlib/Measurements/Load Flow Bus  LConnTagsString=a  ID=bus113  Vbase=150000  Vref=1  Vangle=0  VLF=1  angleLF=0
      settings: AttributesFormatString=|
      | %<ID>
      | %<Vbase>V
      | %<VLF>pu
      | %<angleLF>deg.
      | %<Name>
  bus114 : powerlib/Measurements/Load Flow Bus  LConnTagsString=a  ID=bus114  Vbase=150000  Vref=1  Vangle=0  VLF=1  angleLF=0
      settings: AttributesFormatString=|
      | %<ID>
      | %<Vbase>V
      | %<VLF>pu
      | %<angleLF>deg.
      | %<Name>
  bus115 : powerlib/Measurements/Load Flow Bus  LConnTagsString=a  ID=bus115  Vbase=150000  Vref=1  Vangle=0  VLF=1  angleLF=0
      settings: AttributesFormatString=|
      | %<ID>
      | %<Vbase>V
      | %<VLF>pu
      | %<angleLF>deg.
      | %<Name>
  bus116 : powerlib/Measurements/Load Flow Bus  LConnTagsString=a  ID=bus116  Vbase=150000  Vref=1  Vangle=0  VLF=1  angleLF=0
      settings: AttributesFormatString=|
      | %<ID>
      | %<Vbase>V
      | %<VLF>pu
      | %<angleLF>deg.
      | %<Name>
  bus117 : powerlib/Measurements/Load Flow Bus  LConnTagsString=a  ID=bus117  Vbase=150000  Vref=1  Vangle=0  VLF=1  angleLF=0
      settings: AttributesFormatString=|
      | %<ID>
      | %<Vbase>V
      | %<VLF>pu
      | %<angleLF>deg.
      | %<Name>
  bus118 : powerlib/Measurements/Load Flow Bus  LConnTagsString=a  ID=bus118  Vbase=150000  Vref=1  Vangle=0  VLF=1  angleLF=0
      settings: AttributesFormatString=|
      | %<ID>
      | %<Vbase>V
      | %<VLF>pu
      | %<angleLF>deg.
      | %<Name>
  bus119 : powerlib/Measurements/Load Flow Bus  LConnTagsString=a  ID=bus119  Vbase=150000  Vref=1  Vangle=0  VLF=1  angleLF=0
      settings: AttributesFormatString=|
      | %<ID>
      | %<Vbase>V
      | %<VLF>pu
      | %<angleLF>deg.
      | %<Name>
  bus12 : powerlib/Measurements/Load Flow Bus  LConnTagsString=a  ID=bus12  Vbase=150000  Vref=1  Vangle=0  VLF=1  angleLF=0
      settings: AttributesFormatString=|
      | %<ID>
      | %<Vbase>V
      | %<VLF>pu
      | %<angleLF>deg.
      | %<Name>
  bus120 : powerlib/Measurements/Load Flow Bus  LConnTagsString=a  ID=bus120  Vbase=150000  Vref=1  Vangle=0  VLF=1  angleLF=0
      settings: AttributesFormatString=|
      | %<ID>
      | %<Vbase>V
      | %<VLF>pu
      | %<angleLF>deg.
      | %<Name>
  bus121 : powerlib/Measurements/Load Flow Bus  LConnTagsString=a  ID=bus121  Vbase=400000  Vref=1  Vangle=0  VLF=1  angleLF=0
      settings: AttributesFormatString=|
      | %<ID>
      | %<Vbase>V
      | %<VLF>pu
      | %<angleLF>deg.
      | %<Name>
  bus122 : powerlib/Measurements/Load Flow Bus  LConnTagsString=a  ID=bus122  Vbase=400000  Vref=1  Vangle=0  VLF=1  angleLF=0
      settings: AttributesFormatString=|
      | %<ID>
      | %<Vbase>V
      | %<VLF>pu
      | %<angleLF>deg.
      | %<Name>
  bus123 : powerlib/Measurements/Load Flow Bus  LConnTagsString=a  ID=bus123  Vbase=400000  Vref=1  Vangle=0  VLF=1  angleLF=0
      settings: AttributesFormatString=|
      | %<ID>
      | %<Vbase>V
      | %<VLF>pu
      | %<angleLF>deg.
      | %<Name>
  bus124 : powerlib/Measurements/Load Flow Bus  LConnTagsString=a  ID=bus124  Vbase=400000  Vref=1  Vangle=0  VLF=1  angleLF=0
      settings: AttributesFormatString=|
      | %<ID>
      | %<Vbase>V
      | %<VLF>pu
      | %<angleLF>deg.
      | %<Name>
  bus125 : powerlib/Measurements/Load Flow Bus  LConnTagsString=a  ID=bus125  Vbase=400000  Vref=1  Vangle=0  VLF=1  angleLF=0
      settings: AttributesFormatString=|
      | %<ID>
      | %<Vbase>V
      | %<VLF>pu
      | %<angleLF>deg.
      | %<Name>
  bus126 : powerlib/Measurements/Load Flow Bus  LConnTagsString=a  ID=bus126  Vbase=400000  Vref=1  Vangle=0  VLF=1  angleLF=0
      settings: AttributesFormatString=|
      | %<ID>
      | %<Vbase>V
      | %<VLF>pu
      | %<angleLF>deg.
      | %<Name>
  bus127 : powerlib/Measurements/Load Flow Bus  LConnTagsString=a  ID=bus127  Vbase=400000  Vref=1  Vangle=0  VLF=1  angleLF=0
      settings: AttributesFormatString=|
      | %<ID>
      | %<Vbase>V
      | %<VLF>pu
      | %<angleLF>deg.
      | %<Name>
  bus128 : powerlib/Measurements/Load Flow Bus  LConnTagsString=a  ID=bus128  Vbase=400000  Vref=1  Vangle=0  VLF=1  angleLF=0
      settings: AttributesFormatString=|
      | %<ID>
      | %<Vbase>V
      | %<VLF>pu
      | %<angleLF>deg.
      | %<Name>
  bus129 : powerlib/Measurements/Load Flow Bus  LConnTagsString=a  ID=bus129  Vbase=400000  Vref=1  Vangle=0  VLF=1  angleLF=0
      settings: AttributesFormatString=|
      | %<ID>
      | %<Vbase>V
      | %<VLF>pu
      | %<angleLF>deg.
      | %<Name>
  bus13 : powerlib/Measurements/Load Flow Bus  LConnTagsString=a  ID=bus13  Vbase=150000  Vref=1  Vangle=0  VLF=1  angleLF=0
      settings: AttributesFormatString=|
      | %<ID>
      | %<Vbase>V
      | %<VLF>pu
      | %<angleLF>deg.
      | %<Name>
  bus130 : powerlib/Measurements/Load Flow Bus  LConnTagsString=a  ID=bus130  Vbase=400000  Vref=1  Vangle=0  VLF=1  angleLF=0
      settings: AttributesFormatString=|
      | %<ID>
      | %<Vbase>V
      | %<VLF>pu
      | %<angleLF>deg.
      | %<Name>
  bus131 : powerlib/Measurements/Load Flow Bus  LConnTagsString=a  ID=bus131  Vbase=400000  Vref=1  Vangle=0  VLF=1  angleLF=0
      settings: AttributesFormatString=|
      | %<ID>
      | %<Vbase>V
      | %<VLF>pu
      | %<angleLF>deg.
      | %<Name>
  bus132 : powerlib/Measurements/Load Flow Bus  LConnTagsString=a  ID=bus132  Vbase=400000  Vref=1  Vangle=0  VLF=1  angleLF=0
      settings: AttributesFormatString=|
      | %<ID>
      | %<Vbase>V
      | %<VLF>pu
      | %<angleLF>deg.
      | %<Name>
  bus133 : powerlib/Measurements/Load Flow Bus  LConnTagsString=a  ID=bus133  Vbase=400000  Vref=1  Vangle=0  VLF=1  angleLF=0
      settings: AttributesFormatString=|
      | %<ID>
      | %<Vbase>V
      | %<VLF>pu
      | %<angleLF>deg.
      | %<Name>
  bus134 : powerlib/Measurements/Load Flow Bus  LConnTagsString=a  ID=bus134  Vbase=400000  Vref=1  Vangle=0  VLF=1  angleLF=0
      settings: AttributesFormatString=|
      | %<ID>
      | %<Vbase>V
      | %<VLF>pu
      | %<angleLF>deg.
      | %<Name>
  bus135 : powerlib/Measurements/Load Flow Bus  LConnTagsString=a  ID=bus135  Vbase=400000  Vref=1  Vangle=0  VLF=1  angleLF=0
      settings: AttributesFormatString=|
      | %<ID>
      | %<Vbase>V
      | %<VLF>pu
      | %<angleLF>deg.
      | %<Name>
  bus136 : powerlib/Measurements/Load Flow Bus  LConnTagsString=a  ID=bus136  Vbase=400000  Vref=1  Vangle=0  VLF=1  angleLF=0
      settings: AttributesFormatString=|
      | %<ID>
      | %<Vbase>V
      | %<VLF>pu
      | %<angleLF>deg.
      | %<Name>
  bus137 : powerlib/Measurements/Load Flow Bus  LConnTagsString=a  ID=bus137  Vbase=400000  Vref=1  Vangle=0  VLF=1  angleLF=0
      settings: AttributesFormatString=|
      | %<ID>
      | %<Vbase>V
      | %<VLF>pu
      | %<angleLF>deg.
      | %<Name>
  bus138 : powerlib/Measurements/Load Flow Bus  LConnTagsString=a  ID=bus138  Vbase=400000  Vref=1  Vangle=0  VLF=1  angleLF=0
      settings: AttributesFormatString=|
      | %<ID>
      | %<Vbase>V
      | %<VLF>pu
      | %<angleLF>deg.
      | %<Name>
  bus139 : powerlib/Measurements/Load Flow Bus  LConnTagsString=a  ID=bus139  Vbase=400000  Vref=1  Vangle=0  VLF=1  angleLF=0
      settings: AttributesFormatString=|
      | %<ID>
      | %<Vbase>V
      | %<VLF>pu
      | %<angleLF>deg.
      | %<Name>
  bus14 : powerlib/Measurements/Load Flow Bus  LConnTagsString=a  ID=bus14  Vbase=150000  Vref=1  Vangle=0  VLF=1  angleLF=0
      settings: AttributesFormatString=|
      | %<ID>
      | %<Vbase>V
      | %<VLF>pu
      | %<angleLF>deg.
      | %<Name>
  bus140 : powerlib/Measurements/Load Flow Bus  LConnTagsString=a  ID=bus140  Vbase=400000  Vref=1  Vangle=0  VLF=1  angleLF=0
      settings: AttributesFormatString=|
      | %<ID>
      | %<Vbase>V
      | %<VLF>pu
      | %<angleLF>deg.
      | %<Name>
  bus141 : powerlib/Measurements/Load Flow Bus  LConnTagsString=a  ID=bus141  Vbase=400000  Vref=1  Vangle=0  VLF=1  angleLF=0
      settings: AttributesFormatString=|
      | %<ID>
      | %<Vbase>V
      | %<VLF>pu
      | %<angleLF>deg.
      | %<Name>
  bus142 : powerlib/Measurements/Load Flow Bus  LConnTagsString=a  ID=bus142  Vbase=400000  Vref=1  Vangle=0  VLF=1  angleLF=0
      settings: AttributesFormatString=|
      | %<ID>
      | %<Vbase>V
      | %<VLF>pu
      | %<angleLF>deg.
      | %<Name>
  bus143 : powerlib/Measurements/Load Flow Bus  LConnTagsString=a  ID=bus143  Vbase=400000  Vref=1  Vangle=0  VLF=1  angleLF=0
      settings: AttributesFormatString=|
      | %<ID>
      | %<Vbase>V
      | %<VLF>pu
      | %<angleLF>deg.
      | %<Name>
  bus144 : powerlib/Measurements/Load Flow Bus  LConnTagsString=a  ID=bus144  Vbase=400000  Vref=1  Vangle=0  VLF=1  angleLF=0
      settings: AttributesFormatString=|
      | %<ID>
      | %<Vbase>V
      | %<VLF>pu
      | %<angleLF>deg.
      | %<Name>
  bus145 : powerlib/Measurements/Load Flow Bus  LConnTagsString=a  ID=bus145  Vbase=400000  Vref=1  Vangle=0  VLF=1  angleLF=0
      settings: AttributesFormatString=|
      | %<ID>
      | %<Vbase>V
      | %<VLF>pu
      | %<angleLF>deg.
      | %<Name>
  bus146 : powerlib/Measurements/Load Flow Bus  LConnTagsString=a  ID=bus146  Vbase=150000  Vref=1  Vangle=0  VLF=1  angleLF=0
      settings: AttributesFormatString=|
      | %<ID>
      | %<Vbase>V
      | %<VLF>pu
      | %<angleLF>deg.
      | %<Name>
  bus147 : powerlib/Measurements/Load Flow Bus  LConnTagsString=a  ID=bus147  Vbase=150000  Vref=1  Vangle=0  VLF=1  angleLF=0
      settings: AttributesFormatString=|
      | %<ID>
      | %<Vbase>V
      | %<VLF>pu
      | %<angleLF>deg.
      | %<Name>
  bus148 : powerlib/Measurements/Load Flow Bus  LConnTagsString=a  ID=bus148  Vbase=150000  Vref=1  Vangle=0  VLF=1  angleLF=0
      settings: AttributesFormatString=|
      | %<ID>
      | %<Vbase>V
      | %<VLF>pu
      | %<angleLF>deg.
      | %<Name>
  bus149 : powerlib/Measurements/Load Flow Bus  LConnTagsString=a  ID=bus149  Vbase=150000  Vref=1  Vangle=0  VLF=1  angleLF=0
      settings: AttributesFormatString=|
      | %<ID>
      | %<Vbase>V
      | %<VLF>pu
      | %<angleLF>deg.
      | %<Name>
  bus15 : powerlib/Measurements/Load Flow Bus  LConnTagsString=a  ID=bus15  Vbase=150000  Vref=1  Vangle=0  VLF=1  angleLF=0
      settings: AttributesFormatString=|
      | %<ID>
      | %<Vbase>V
      | %<VLF>pu
      | %<angleLF>deg.
      | %<Name>
  bus150 : powerlib/Measurements/Load Flow Bus  LConnTagsString=a  ID=bus150  Vbase=150000  Vref=1  Vangle=0  VLF=1  angleLF=0
      settings: AttributesFormatString=|
      | %<ID>
      | %<Vbase>V
      | %<VLF>pu
      | %<angleLF>deg.
      | %<Name>
  bus151 : powerlib/Measurements/Load Flow Bus  LConnTagsString=a  ID=bus151  Vbase=150000  Vref=1  Vangle=0  VLF=1  angleLF=0
      settings: AttributesFormatString=|
      | %<ID>
      | %<Vbase>V
      | %<VLF>pu
      | %<angleLF>deg.
      | %<Name>
  bus152 : powerlib/Measurements/Load Flow Bus  LConnTagsString=a  ID=bus152  Vbase=150000  Vref=1  Vangle=0  VLF=1  angleLF=0
      settings: AttributesFormatString=|
      | %<ID>
      | %<Vbase>V
      | %<VLF>pu
      | %<angleLF>deg.
      | %<Name>
  bus153 : powerlib/Measurements/Load Flow Bus  LConnTagsString=a  ID=bus153  Vbase=150000  Vref=1  Vangle=0  VLF=1  angleLF=0
      settings: AttributesFormatString=|
      | %<ID>
      | %<Vbase>V
      | %<VLF>pu
      | %<angleLF>deg.
      | %<Name>
  bus154 : powerlib/Measurements/Load Flow Bus  LConnTagsString=a  ID=bus154  Vbase=150000  Vref=1  Vangle=0  VLF=1  angleLF=0
      settings: AttributesFormatString=|
      | %<ID>
      | %<Vbase>V
      | %<VLF>pu
      | %<angleLF>deg.
      | %<Name>
  bus155 : powerlib/Measurements/Load Flow Bus  LConnTagsString=a  ID=bus155  Vbase=150000  Vref=1  Vangle=0  VLF=1  angleLF=0
      settings: AttributesFormatString=|
      | %<ID>
      | %<Vbase>V
      | %<VLF>pu
      | %<angleLF>deg.
      | %<Name>
  bus156 : powerlib/Measurements/Load Flow Bus  LConnTagsString=a  ID=bus156  Vbase=150000  Vref=1  Vangle=0  VLF=1  angleLF=0
      settings: AttributesFormatString=|
      | %<ID>
      | %<Vbase>V
      | %<VLF>pu
      | %<angleLF>deg.
      | %<Name>
  bus157 : powerlib/Measurements/Load Flow Bus  LConnTagsString=a  ID=bus157  Vbase=150000  Vref=1  Vangle=0  VLF=1  angleLF=0
      settings: AttributesFormatString=|
      | %<ID>
      | %<Vbase>V
      | %<VLF>pu
      | %<angleLF>deg.
      | %<Name>
  bus158 : powerlib/Measurements/Load Flow Bus  LConnTagsString=a  ID=bus158  Vbase=150000  Vref=1  Vangle=0  VLF=1  angleLF=0
      settings: AttributesFormatString=|
      | %<ID>
      | %<Vbase>V
      | %<VLF>pu
      | %<angleLF>deg.
      | %<Name>
  bus159 : powerlib/Measurements/Load Flow Bus  LConnTagsString=a  ID=bus159  Vbase=150000  Vref=1  Vangle=0  VLF=1  angleLF=0
      settings: AttributesFormatString=|
      | %<ID>
      | %<Vbase>V
      | %<VLF>pu
      | %<angleLF>deg.
      | %<Name>
  bus16 : powerlib/Measurements/Load Flow Bus  LConnTagsString=a  ID=bus16  Vbase=150000  Vref=1  Vangle=0  VLF=1  angleLF=0
      settings: AttributesFormatString=|
      | %<ID>
      | %<Vbase>V
      | %<VLF>pu
      | %<angleLF>deg.
      | %<Name>
  bus160 : powerlib/Measurements/Load Flow Bus  LConnTagsString=a  ID=bus160  Vbase=150000  Vref=1  Vangle=0  VLF=1  angleLF=0
      settings: AttributesFormatString=|
      | %<ID>
      | %<Vbase>V
      | %<VLF>pu
      | %<angleLF>deg.
      | %<Name>
  bus161 : powerlib/Measurements/Load Flow Bus  LConnTagsString=a  ID=bus161  Vbase=150000  Vref=1  Vangle=0  VLF=1  angleLF=0
      settings: AttributesFormatString=|
      | %<ID>
      | %<Vbase>V
      | %<VLF>pu
      | %<angleLF>deg.
      | %<Name>
  bus162 : powerlib/Measurements/Load Flow Bus  LConnTagsString=a  ID=bus162  Vbase=150000  Vref=1  Vangle=0  VLF=1  angleLF=0
      settings: AttributesFormatString=|
      | %<ID>
      | %<Vbase>V
      | %<VLF>pu
      | %<angleLF>deg.
      | %<Name>
  bus163 : powerlib/Measurements/Load Flow Bus  LConnTagsString=a  ID=bus163  Vbase=150000  Vref=1  Vangle=0  VLF=1  angleLF=0
      settings: AttributesFormatString=|
      | %<ID>
      | %<Vbase>V
      | %<VLF>pu
      | %<angleLF>deg.
      | %<Name>
  bus164 : powerlib/Measurements/Load Flow Bus  LConnTagsString=a  ID=bus164  Vbase=150000  Vref=1  Vangle=0  VLF=1  angleLF=0
      settings: AttributesFormatString=|
      | %<ID>
      | %<Vbase>V
      | %<VLF>pu
      | %<angleLF>deg.
      | %<Name>
  bus165 : powerlib/Measurements/Load Flow Bus  LConnTagsString=a  ID=bus165  Vbase=150000  Vref=1  Vangle=0  VLF=1  angleLF=0
      settings: AttributesFormatString=|
      | %<ID>
      | %<Vbase>V
      | %<VLF>pu
      | %<angleLF>deg.
      | %<Name>
  bus166 : powerlib/Measurements/Load Flow Bus  LConnTagsString=a  ID=bus166  Vbase=150000  Vref=1  Vangle=0  VLF=1  angleLF=0
      settings: AttributesFormatString=|
      | %<ID>
      | %<Vbase>V
      | %<VLF>pu
      | %<angleLF>deg.
      | %<Name>
  bus167 : powerlib/Measurements/Load Flow Bus  LConnTagsString=a  ID=bus167  Vbase=150000  Vref=1  Vangle=0  VLF=1  angleLF=0
      settings: AttributesFormatString=|
      | %<ID>
      | %<Vbase>V
      | %<VLF>pu
      | %<angleLF>deg.
      | %<Name>
  bus168 : powerlib/Measurements/Load Flow Bus  LConnTagsString=a  ID=bus168  Vbase=150000  Vref=1  Vangle=0  VLF=1  angleLF=0
      settings: AttributesFormatString=|
      | %<ID>
      | %<Vbase>V
      | %<VLF>pu
      | %<angleLF>deg.
      | %<Name>
  bus169 : powerlib/Measurements/Load Flow Bus  LConnTagsString=a  ID=bus169  Vbase=150000  Vref=1  Vangle=0  VLF=1  angleLF=0
      settings: AttributesFormatString=|
      | %<ID>
      | %<Vbase>V
      | %<VLF>pu
      | %<angleLF>deg.
      | %<Name>
  bus17 : powerlib/Measurements/Load Flow Bus  LConnTagsString=a  ID=bus17  Vbase=150000  Vref=1  Vangle=0  VLF=1  angleLF=0
      settings: AttributesFormatString=|
      | %<ID>
      | %<Vbase>V
      | %<VLF>pu
      | %<angleLF>deg.
      | %<Name>
  bus170 : powerlib/Measurements/Load Flow Bus  LConnTagsString=a  ID=bus170  Vbase=150000  Vref=1  Vangle=0  VLF=1  angleLF=0
      settings: AttributesFormatString=|
      | %<ID>
      | %<Vbase>V
      | %<VLF>pu
      | %<angleLF>deg.
      | %<Name>
  bus171 : powerlib/Measurements/Load Flow Bus  LConnTagsString=a  ID=bus171  Vbase=150000  Vref=1  Vangle=0  VLF=1  angleLF=0
      settings: AttributesFormatString=|
      | %<ID>
      | %<Vbase>V
      | %<VLF>pu
      | %<angleLF>deg.
      | %<Name>
  bus172 : powerlib/Measurements/Load Flow Bus  LConnTagsString=a  ID=bus172  Vbase=150000  Vref=1  Vangle=0  VLF=1  angleLF=0
      settings: AttributesFormatString=|
      | %<ID>
      | %<Vbase>V
      | %<VLF>pu
      | %<angleLF>deg.
      | %<Name>
  bus173 : powerlib/Measurements/Load Flow Bus  LConnTagsString=a  ID=bus173  Vbase=150000  Vref=1  Vangle=0  VLF=1  angleLF=0
      settings: AttributesFormatString=|
      | %<ID>
      | %<Vbase>V
      | %<VLF>pu
      | %<angleLF>deg.
      | %<Name>
  bus174 : powerlib/Measurements/Load Flow Bus  LConnTagsString=a  ID=bus174  Vbase=150000  Vref=1  Vangle=0  VLF=1  angleLF=0
      settings: AttributesFormatString=|
      | %<ID>
      | %<Vbase>V
      | %<VLF>pu
      | %<angleLF>deg.
      | %<Name>
  bus175 : powerlib/Measurements/Load Flow Bus  LConnTagsString=a  ID=bus175  Vbase=150000  Vref=1  Vangle=0  VLF=1  angleLF=0
      settings: AttributesFormatString=|
      | %<ID>
      | %<Vbase>V
      | %<VLF>pu
      | %<angleLF>deg.
      | %<Name>
  bus176 : powerlib/Measurements/Load Flow Bus  LConnTagsString=a  ID=bus176  Vbase=150000  Vref=1  Vangle=0  VLF=1  angleLF=0
      settings: AttributesFormatString=|
      | %<ID>
      | %<Vbase>V
      | %<VLF>pu
      | %<angleLF>deg.
      | %<Name>
  bus177 : powerlib/Measurements/Load Flow Bus  LConnTagsString=a  ID=bus177  Vbase=150000  Vref=1  Vangle=0  VLF=1  angleLF=0
      settings: AttributesFormatString=|
      | %<ID>
      | %<Vbase>V
      | %<VLF>pu
      | %<angleLF>deg.
      | %<Name>
  bus178 : powerlib/Measurements/Load Flow Bus  LConnTagsString=a  ID=bus178  Vbase=150000  Vref=1  Vangle=0  VLF=1  angleLF=0
      settings: AttributesFormatString=|
      | %<ID>
      | %<Vbase>V
      | %<VLF>pu
      | %<angleLF>deg.
      | %<Name>
  bus179 : powerlib/Measurements/Load Flow Bus  LConnTagsString=a  ID=bus179  Vbase=150000  Vref=1  Vangle=0  VLF=1  angleLF=0
      settings: AttributesFormatString=|
      | %<ID>
      | %<Vbase>V
      | %<VLF>pu
      | %<angleLF>deg.
      | %<Name>
  bus18 : powerlib/Measurements/Load Flow Bus  LConnTagsString=a  ID=bus18  Vbase=150000  Vref=1  Vangle=0  VLF=1  angleLF=0
      settings: AttributesFormatString=|
      | %<ID>
      | %<Vbase>V
      | %<VLF>pu
      | %<angleLF>deg.
      | %<Name>
  bus180 : powerlib/Measurements/Load Flow Bus  LConnTagsString=a  ID=bus180  Vbase=150000  Vref=1  Vangle=0  VLF=1  angleLF=0
      settings: AttributesFormatString=|
      | %<ID>
      | %<Vbase>V
      | %<VLF>pu
      | %<angleLF>deg.
      | %<Name>
  bus181 : powerlib/Measurements/Load Flow Bus  LConnTagsString=a  ID=bus181  Vbase=150000  Vref=1  Vangle=0  VLF=1  angleLF=0
      settings: AttributesFormatString=|
      | %<ID>
      | %<Vbase>V
      | %<VLF>pu
      | %<angleLF>deg.
      | %<Name>
  bus182 : powerlib/Measurements/Load Flow Bus  LConnTagsString=a  ID=bus182  Vbase=150000  Vref=1  Vangle=0  VLF=1  angleLF=0
      settings: AttributesFormatString=|
      | %<ID>
      | %<Vbase>V
      | %<VLF>pu
      | %<angleLF>deg.
      | %<Name>
  bus183 : powerlib/Measurements/Load Flow Bus  LConnTagsString=a  ID=bus183  Vbase=150000  Vref=1  Vangle=0  VLF=1  angleLF=0
      settings: AttributesFormatString=|
      | %<ID>
      | %<Vbase>V
      | %<VLF>pu
      | %<angleLF>deg.
      | %<Name>
  bus184 : powerlib/Measurements/Load Flow Bus  LConnTagsString=a  ID=bus184  Vbase=150000  Vref=1  Vangle=0  VLF=1  angleLF=0
      settings: AttributesFormatString=|
      | %<ID>
      | %<Vbase>V
      | %<VLF>pu
      | %<angleLF>deg.
      | %<Name>
  bus185 : powerlib/Measurements/Load Flow Bus  LConnTagsString=a  ID=bus185  Vbase=150000  Vref=1  Vangle=0  VLF=1  angleLF=0
      settings: AttributesFormatString=|
      | %<ID>
      | %<Vbase>V
      | %<VLF>pu
      | %<angleLF>deg.
      | %<Name>
  bus186 : powerlib/Measurements/Load Flow Bus  LConnTagsString=a  ID=bus186  Vbase=150000  Vref=1  Vangle=0  VLF=1  angleLF=0
      settings: AttributesFormatString=|
      | %<ID>
      | %<Vbase>V
      | %<VLF>pu
      | %<angleLF>deg.
      | %<Name>
  bus187 : powerlib/Measurements/Load Flow Bus  LConnTagsString=a  ID=bus187  Vbase=150000  Vref=1  Vangle=0  VLF=1  angleLF=0
      settings: AttributesFormatString=|
      | %<ID>
      | %<Vbase>V
      | %<VLF>pu
      | %<angleLF>deg.
      | %<Name>
  bus188 : powerlib/Measurements/Load Flow Bus  LConnTagsString=a  ID=bus188  Vbase=150000  Vref=1  Vangle=0  VLF=1  angleLF=0
      settings: AttributesFormatString=|
      | %<ID>
      | %<Vbase>V
      | %<VLF>pu
      | %<angleLF>deg.
      | %<Name>
  bus189 : powerlib/Measurements/Load Flow Bus  LConnTagsString=a  ID=bus189  Vbase=150000  Vref=1  Vangle=0  VLF=1  angleLF=0
      settings: AttributesFormatString=|
      | %<ID>
      | %<Vbase>V
      | %<VLF>pu
      | %<angleLF>deg.
      | %<Name>
  bus19 : powerlib/Measurements/Load Flow Bus  LConnTagsString=a  ID=bus19  Vbase=150000  Vref=1  Vangle=0  VLF=1  angleLF=0
      settings: AttributesFormatString=|
      | %<ID>
      | %<Vbase>V
      | %<VLF>pu
      | %<angleLF>deg.
      | %<Name>
  bus190 : powerlib/Measurements/Load Flow Bus  LConnTagsString=a  ID=bus190  Vbase=150000  Vref=1  Vangle=0  VLF=1  angleLF=0
      settings: AttributesFormatString=|
      | %<ID>
      | %<Vbase>V
      | %<VLF>pu
      | %<angleLF>deg.
      | %<Name>
  bus191 : powerlib/Measurements/Load Flow Bus  LConnTagsString=a  ID=bus191  Vbase=150000  Vref=1  Vangle=0  VLF=1  angleLF=0
      settings: AttributesFormatString=|
      | %<ID>
      | %<Vbase>V
      | %<VLF>pu
      | %<angleLF>deg.
      | %<Name>
  bus192 : powerlib/Measurements/Load Flow Bus  LConnTagsString=a  ID=bus192  Vbase=150000  Vref=1  Vangle=0  VLF=1  angleLF=0
      settings: AttributesFormatString=|
      | %<ID>
      | %<Vbase>V
      | %<VLF>pu
      | %<angleLF>deg.
      | %<Name>
  bus193 : powerlib/Measurements/Load Flow Bus  LConnTagsString=a  ID=bus193  Vbase=150000  Vref=1  Vangle=0  VLF=1  angleLF=0
      settings: AttributesFormatString=|
      | %<ID>
      | %<Vbase>V
      | %<VLF>pu
      | %<angleLF>deg.
      | %<Name>
  bus194 : powerlib/Measurements/Load Flow Bus  LConnTagsString=a  ID=bus194  Vbase=150000  Vref=1  Vangle=0  VLF=1  angleLF=0
      settings: AttributesFormatString=|
      | %<ID>
      | %<Vbase>V
      | %<VLF>pu
      | %<angleLF>deg.
      | %<Name>
  bus195 : powerlib/Measurements/Load Flow Bus  LConnTagsString=a  ID=bus195  Vbase=150000  Vref=1  Vangle=0  VLF=1  angleLF=0
      settings: AttributesFormatString=|
      | %<ID>
      | %<Vbase>V
      | %<VLF>pu
      | %<angleLF>deg.
      | %<Name>
  bus196 : powerlib/Measurements/Load Flow Bus  LConnTagsString=a  ID=bus196  Vbase=150000  Vref=1  Vangle=0  VLF=1  angleLF=0
      settings: AttributesFormatString=|
      | %<ID>
      | %<Vbase>V
      | %<VLF>pu
      | %<angleLF>deg.
      | %<Name>
  bus197 : powerlib/Measurements/Load Flow Bus  LConnTagsString=a  ID=bus197  Vbase=150000  Vref=1  Vangle=0  VLF=1  angleLF=0
      settings: AttributesFormatString=|
      | %<ID>
      | %<Vbase>V
      | %<VLF>pu
      | %<angleLF>deg.
      | %<Name>
  bus198 : powerlib/Measurements/Load Flow Bus  LConnTagsString=a  ID=bus198  Vbase=150000  Vref=1  Vangle=0  VLF=1  angleLF=0
      settings: AttributesFormatString=|
      | %<ID>
      | %<Vbase>V
      | %<VLF>pu
      | %<angleLF>deg.
      | %<Name>
  bus199 : powerlib/Measurements/Load Flow Bus  LConnTagsString=a  ID=bus199  Vbase=150000  Vref=1  Vangle=0  VLF=1  angleLF=0
      settings: AttributesFormatString=|
      | %<ID>
      | %<Vbase>V
      | %<VLF>pu
      | %<angleLF>deg.
      | %<Name>
  bus2 : powerlib/Measurements/Load Flow Bus  LConnTagsString=a  ID=bus2  Vbase=150000  Vref=1  Vangle=0  VLF=1  angleLF=0
      settings: AttributesFormatString=|
      | %<ID>
      | %<Vbase>V
      | %<VLF>pu
      | %<angleLF>deg.
      | %<Name>
  bus20 : powerlib/Measurements/Load Flow Bus  LConnTagsString=a  ID=bus20  Vbase=150000  Vref=1  Vangle=0  VLF=1  angleLF=0
      settings: AttributesFormatString=|
      | %<ID>
      | %<Vbase>V
      | %<VLF>pu
      | %<angleLF>deg.
      | %<Name>
  bus200 : powerlib/Measurements/Load Flow Bus  LConnTagsString=a  ID=bus200  Vbase=150000  Vref=1  Vangle=0  VLF=1  angleLF=0
      settings: AttributesFormatString=|
      | %<ID>
      | %<Vbase>V
      | %<VLF>pu
      | %<angleLF>deg.
      | %<Name>
  bus201 : powerlib/Measurements/Load Flow Bus  LConnTagsString=a  ID=bus201  Vbase=150000  Vref=1  Vangle=0  VLF=1  angleLF=0
      settings: AttributesFormatString=|
      | %<ID>
      | %<Vbase>V
      | %<VLF>pu
      | %<angleLF>deg.
      | %<Name>
  bus202 : powerlib/Measurements/Load Flow Bus  LConnTagsString=a  ID=bus202  Vbase=150000  Vref=1  Vangle=0  VLF=1  angleLF=0
      settings: AttributesFormatString=|
      | %<ID>
      | %<Vbase>V
      | %<VLF>pu
      | %<angleLF>deg.
      | %<Name>
  bus203 : powerlib/Measurements/Load Flow Bus  LConnTagsString=a  ID=bus203  Vbase=150000  Vref=1  Vangle=0  VLF=1  angleLF=0
      settings: AttributesFormatString=|
      | %<ID>
      | %<Vbase>V
      | %<VLF>pu
      | %<angleLF>deg.
      | %<Name>
  bus204 : powerlib/Measurements/Load Flow Bus  LConnTagsString=a  ID=bus204  Vbase=150000  Vref=1  Vangle=0  VLF=1  angleLF=0
      settings: AttributesFormatString=|
      | %<ID>
      | %<Vbase>V
      | %<VLF>pu
      | %<angleLF>deg.
      | %<Name>
  bus205 : powerlib/Measurements/Load Flow Bus  LConnTagsString=a  ID=bus205  Vbase=150000  Vref=1  Vangle=0  VLF=1  angleLF=0
      settings: AttributesFormatString=|
      | %<ID>
      | %<Vbase>V
      | %<VLF>pu
      | %<angleLF>deg.
      | %<Name>
  bus206 : powerlib/Measurements/Load Flow Bus  LConnTagsString=a  ID=bus206  Vbase=150000  Vref=1  Vangle=0  VLF=1  angleLF=0
      settings: AttributesFormatString=|
      | %<ID>
      | %<Vbase>V
      | %<VLF>pu
      | %<angleLF>deg.
      | %<Name>
  bus207 : powerlib/Measurements/Load Flow Bus  LConnTagsString=a  ID=bus207  Vbase=150000  Vref=1  Vangle=0  VLF=1  angleLF=0
      settings: AttributesFormatString=|
      | %<ID>
      | %<Vbase>V
      | %<VLF>pu
      | %<angleLF>deg.
      | %<Name>
  bus208 : powerlib/Measurements/Load Flow Bus  LConnTagsString=a  ID=bus208  Vbase=150000  Vref=1  Vangle=0  VLF=1  angleLF=0
      settings: AttributesFormatString=|
      | %<ID>
      | %<Vbase>V
      | %<VLF>pu
      | %<angleLF>deg.
      | %<Name>
  bus209 : powerlib/Measurements/Load Flow Bus  LConnTagsString=a  ID=bus209  Vbase=150000  Vref=1  Vangle=0  VLF=1  angleLF=0
      settings: AttributesFormatString=|
      | %<ID>
      | %<Vbase>V
      | %<VLF>pu
      | %<angleLF>deg.
      | %<Name>
  bus21 : powerlib/Measurements/Load Flow Bus  LConnTagsString=a  ID=bus21  Vbase=150000  Vref=1  Vangle=0  VLF=1  angleLF=0
      settings: AttributesFormatString=|
      | %<ID>
      | %<Vbase>V
      | %<VLF>pu
      | %<angleLF>deg.
      | %<Name>
  bus210 : powerlib/Measurements/Load Flow Bus  LConnTagsString=a  ID=bus210  Vbase=150000  Vref=1  Vangle=0  VLF=1  angleLF=0
      settings: AttributesFormatString=|
      | %<ID>
      | %<Vbase>V
      | %<VLF>pu
      | %<angleLF>deg.
      | %<Name>
  bus211 : powerlib/Measurements/Load Flow Bus  LConnTagsString=a  ID=bus211  Vbase=150000  Vref=1  Vangle=0  VLF=1  angleLF=0
      settings: AttributesFormatString=|
      | %<ID>
      | %<Vbase>V
      | %<VLF>pu
      | %<angleLF>deg.
      | %<Name>
  bus212 : powerlib/Measurements/Load Flow Bus  LConnTagsString=a  ID=bus212  Vbase=150000  Vref=1  Vangle=0  VLF=1  angleLF=0
      settings: AttributesFormatString=|
      | %<ID>
      | %<Vbase>V
      | %<VLF>pu
      | %<angleLF>deg.
      | %<Name>
  bus213 : powerlib/Measurements/Load Flow Bus  LConnTagsString=a  ID=bus213  Vbase=150000  Vref=1  Vangle=0  VLF=1  angleLF=0
      settings: AttributesFormatString=|
      | %<ID>
      | %<Vbase>V
      | %<VLF>pu
      | %<angleLF>deg.
      | %<Name>
  bus214 : powerlib/Measurements/Load Flow Bus  LConnTagsString=a  ID=bus214  Vbase=150000  Vref=1  Vangle=0  VLF=1  angleLF=0
      settings: AttributesFormatString=|
      | %<ID>
      | %<Vbase>V
      | %<VLF>pu
      | %<angleLF>deg.
      | %<Name>
  bus215 : powerlib/Measurements/Load Flow Bus  LConnTagsString=a  ID=bus215  Vbase=150000  Vref=1  Vangle=0  VLF=1  angleLF=0
      settings: AttributesFormatString=|
      | %<ID>
      | %<Vbase>V
      | %<VLF>pu
      | %<angleLF>deg.
      | %<Name>
  bus216 : powerlib/Measurements/Load Flow Bus  LConnTagsString=a  ID=bus216  Vbase=150000  Vref=1  Vangle=0  VLF=1  angleLF=0
      settings: AttributesFormatString=|
      | %<ID>
      | %<Vbase>V
      | %<VLF>pu
      | %<angleLF>deg.
      | %<Name>
  bus217 : powerlib/Measurements/Load Flow Bus  LConnTagsString=a  ID=bus217  Vbase=150000  Vref=1  Vangle=0  VLF=1  angleLF=0
      settings: AttributesFormatString=|
      | %<ID>
      | %<Vbase>V
      | %<VLF>pu
      | %<angleLF>deg.
      | %<Name>
  bus218 : powerlib/Measurements/Load Flow Bus  LConnTagsString=a  ID=bus218  Vbase=150000  Vref=1  Vangle=0  VLF=1  angleLF=0
      settings: AttributesFormatString=|
      | %<ID>
      | %<Vbase>V
      | %<VLF>pu
      | %<angleLF>deg.
      | %<Name>
  bus219 : powerlib/Measurements/Load Flow Bus  LConnTagsString=a  ID=bus219  Vbase=150000  Vref=1  Vangle=0  VLF=1  angleLF=0
      settings: AttributesFormatString=|
      | %<ID>
      | %<Vbase>V
      | %<VLF>pu
      | %<angleLF>deg.
      | %<Name>
  bus22 : powerlib/Measurements/Load Flow Bus  LConnTagsString=a  ID=bus22  Vbase=150000  Vref=1  Vangle=0  VLF=1  angleLF=0
      settings: AttributesFormatString=|
      | %<ID>
      | %<Vbase>V
      | %<VLF>pu
      | %<angleLF>deg.
      | %<Name>
  bus220 : powerlib/Measurements/Load Flow Bus  LConnTagsString=a  ID=bus220  Vbase=150000  Vref=1  Vangle=0  VLF=1  angleLF=0
      settings: AttributesFormatString=|
      | %<ID>
      | %<Vbase>V
      | %<VLF>pu
      | %<angleLF>deg.
      | %<Name>
  bus221 : powerlib/Measurements/Load Flow Bus  LConnTagsString=a  ID=bus221  Vbase=150000  Vref=1  Vangle=0  VLF=1  angleLF=0
      settings: AttributesFormatString=|
      | %<ID>
      | %<Vbase>V
      | %<VLF>pu
      | %<angleLF>deg.
      | %<Name>
  bus222 : powerlib/Measurements/Load Flow Bus  LConnTagsString=a  ID=bus222  Vbase=150000  Vref=1  Vangle=0  VLF=1  angleLF=0
      settings: AttributesFormatString=|
      | %<ID>
      | %<Vbase>V
      | %<VLF>pu
      | %<angleLF>deg.
      | %<Name>
  bus223 : powerlib/Measurements/Load Flow Bus  LConnTagsString=a  ID=bus223  Vbase=150000  Vref=1  Vangle=0  VLF=1  angleLF=0
      settings: AttributesFormatString=|
      | %<ID>
      | %<Vbase>V
      | %<VLF>pu
      | %<angleLF>deg.
      | %<Name>
  bus224 : powerlib/Measurements/Load Flow Bus  LConnTagsString=a  ID=bus224  Vbase=150000  Vref=1  Vangle=0  VLF=1  angleLF=0
      settings: AttributesFormatString=|
      | %<ID>
      | %<Vbase>V
      | %<VLF>pu
      | %<angleLF>deg.
      | %<Name>
  bus225 : powerlib/Measurements/Load Flow Bus  LConnTagsString=a  ID=bus225  Vbase=150000  Vref=1  Vangle=0  VLF=1  angleLF=0
      settings: AttributesFormatString=|
      | %<ID>
      | %<Vbase>V
      | %<VLF>pu
      | %<angleLF>deg.
      | %<Name>
  bus226 : powerlib/Measurements/Load Flow Bus  LConnTagsString=a  ID=bus226  Vbase=150000  Vref=1  Vangle=0  VLF=1  angleLF=0
      settings: AttributesFormatString=|
      | %<ID>
      | %<Vbase>V
      | %<VLF>pu
      | %<angleLF>deg.
      | %<Name>
  bus227 : powerlib/Measurements/Load Flow Bus  LConnTagsString=a  ID=bus227  Vbase=150000  Vref=1  Vangle=0  VLF=1  angleLF=0
      settings: AttributesFormatString=|
      | %<ID>
      | %<Vbase>V
      | %<VLF>pu
      | %<angleLF>deg.
      | %<Name>
  bus228 : powerlib/Measurements/Load Flow Bus  LConnTagsString=a  ID=bus228  Vbase=150000  Vref=1  Vangle=0  VLF=1  angleLF=0
      settings: AttributesFormatString=|
      | %<ID>
      | %<Vbase>V
      | %<VLF>pu
      | %<angleLF>deg.
      | %<Name>
  bus229 : powerlib/Measurements/Load Flow Bus  LConnTagsString=a  ID=bus229  Vbase=150000  Vref=1  Vangle=0  VLF=1  angleLF=0
      settings: AttributesFormatString=|
      | %<ID>
      | %<Vbase>V
      | %<VLF>pu
      | %<angleLF>deg.
      | %<Name>
  bus23 : powerlib/Measurements/Load Flow Bus  LConnTagsString=a  ID=bus23  Vbase=150000  Vref=1  Vangle=0  VLF=1  angleLF=0
      settings: AttributesFormatString=|
      | %<ID>
      | %<Vbase>V
      | %<VLF>pu
      | %<angleLF>deg.
      | %<Name>
  bus230 : powerlib/Measurements/Load Flow Bus  LConnTagsString=a  ID=bus230  Vbase=150000  Vref=1  Vangle=0  VLF=1  angleLF=0
      settings: AttributesFormatString=|
      | %<ID>
      | %<Vbase>V
      | %<VLF>pu
      | %<angleLF>deg.
      | %<Name>
  bus231 : powerlib/Measurements/Load Flow Bus  LConnTagsString=a  ID=bus231  Vbase=150000  Vref=1  Vangle=0  VLF=1  angleLF=0
      settings: AttributesFormatString=|
      | %<ID>
      | %<Vbase>V
      | %<VLF>pu
      | %<angleLF>deg.
      | %<Name>
  bus232 : powerlib/Measurements/Load Flow Bus  LConnTagsString=a  ID=bus232  Vbase=150000  Vref=1  Vangle=0  VLF=1  angleLF=0
      settings: AttributesFormatString=|
      | %<ID>
      | %<Vbase>V
      | %<VLF>pu
      | %<angleLF>deg.
      | %<Name>
  bus233 : powerlib/Measurements/Load Flow Bus  LConnTagsString=a  ID=bus233  Vbase=150000  Vref=1  Vangle=0  VLF=1  angleLF=0
      settings: AttributesFormatString=|
      | %<ID>
      | %<Vbase>V
      | %<VLF>pu
      | %<angleLF>deg.
      | %<Name>
  bus234 : powerlib/Measurements/Load Flow Bus  LConnTagsString=a  ID=bus234  Vbase=150000  Vref=1  Vangle=0  VLF=1  angleLF=0
      settings: AttributesFormatString=|
      | %<ID>
      | %<Vbase>V
      | %<VLF>pu
      | %<angleLF>deg.
      | %<Name>
  bus235 : powerlib/Measurements/Load Flow Bus  LConnTagsString=a  ID=bus235  Vbase=150000  Vref=1  Vangle=0  VLF=1  angleLF=0
      settings: AttributesFormatString=|
      | %<ID>
      | %<Vbase>V
      | %<VLF>pu
      | %<angleLF>deg.
      | %<Name>
  bus236 : powerlib/Measurements/Load Flow Bus  LConnTagsString=a  ID=bus236  Vbase=150000  Vref=1  Vangle=0  VLF=1  angleLF=0
      settings: AttributesFormatString=|
      | %<ID>
      | %<Vbase>V
      | %<VLF>pu
      | %<angleLF>deg.
      | %<Name>
  bus237 : powerlib/Measurements/Load Flow Bus  LConnTagsString=a  ID=bus237  Vbase=150000  Vref=1  Vangle=0  VLF=1  angleLF=0
      settings: AttributesFormatString=|
      | %<ID>
      | %<Vbase>V
      | %<VLF>pu
      | %<angleLF>deg.
      | %<Name>
  bus238 : powerlib/Measurements/Load Flow Bus  LConnTagsString=a  ID=bus238  Vbase=150000  Vref=1  Vangle=0  VLF=1  angleLF=0
      settings: AttributesFormatString=|
      | %<ID>
      | %<Vbase>V
      | %<VLF>pu
      | %<angleLF>deg.
      | %<Name>
  bus239 : powerlib/Measurements/Load Flow Bus  LConnTagsString=a  ID=bus239  Vbase=150000  Vref=1  Vangle=0  VLF=1  angleLF=0
      settings: AttributesFormatString=|
      | %<ID>
      | %<Vbase>V
      | %<VLF>pu
      | %<angleLF>deg.
      | %<Name>
  bus24 : powerlib/Measurements/Load Flow Bus  LConnTagsString=a  ID=bus24  Vbase=150000  Vref=1  Vangle=0  VLF=1  angleLF=0
      settings: AttributesFormatString=|
      | %<ID>
      | %<Vbase>V
      | %<VLF>pu
      | %<angleLF>deg.
      | %<Name>
  bus240 : powerlib/Measurements/Load Flow Bus  LConnTagsString=a  ID=bus240  Vbase=150000  Vref=1  Vangle=0  VLF=1  angleLF=0
      settings: AttributesFormatString=|
      | %<ID>
      | %<Vbase>V
      | %<VLF>pu
      | %<angleLF>deg.
      | %<Name>
  bus241 : powerlib/Measurements/Load Flow Bus  LConnTagsString=a  ID=bus241  Vbase=150000  Vref=1  Vangle=0  VLF=1  angleLF=0
      settings: AttributesFormatString=|
      | %<ID>
      | %<Vbase>V
      | %<VLF>pu
      | %<angleLF>deg.
      | %<Name>
  bus242 : powerlib/Measurements/Load Flow Bus  LConnTagsString=a  ID=bus242  Vbase=150000  Vref=1  Vangle=0  VLF=1  angleLF=0
      settings: AttributesFormatString=|
      | %<ID>
      | %<Vbase>V
      | %<VLF>pu
      | %<angleLF>deg.
      | %<Name>
  bus243 : powerlib/Measurements/Load Flow Bus  LConnTagsString=a  ID=bus243  Vbase=150000  Vref=1  Vangle=0  VLF=1  angleLF=0
      settings: AttributesFormatString=|
      | %<ID>
      | %<Vbase>V
      | %<VLF>pu
      | %<angleLF>deg.
      | %<Name>
  bus244 : powerlib/Measurements/Load Flow Bus  LConnTagsString=a  ID=bus244  Vbase=150000  Vref=1  Vangle=0  VLF=1  angleLF=0
      settings: AttributesFormatString=|
      | %<ID>
      | %<Vbase>V
      | %<VLF>pu
      | %<angleLF>deg.
      | %<Name>
  bus245 : powerlib/Measurements/Load Flow Bus  LConnTagsString=a  ID=bus245  Vbase=150000  Vref=1  Vangle=0  VLF=1  angleLF=0
      settings: AttributesFormatString=|
      | %<ID>
      | %<Vbase>V
      | %<VLF>pu
      | %<angleLF>deg.
      | %<Name>
  bus246 : powerlib/Measurements/Load Flow Bus  LConnTagsString=a  ID=bus246  Vbase=150000  Vref=1  Vangle=0  VLF=1  angleLF=0
      settings: AttributesFormatString=|
      | %<ID>
      | %<Vbase>V
      | %<VLF>pu
      | %<angleLF>deg.
      | %<Name>
  bus247 : powerlib/Measurements/Load Flow Bus  LConnTagsString=a  ID=bus247  Vbase=150000  Vref=1  Vangle=0  VLF=1  angleLF=0
      settings: AttributesFormatString=|
      | %<ID>
      | %<Vbase>V
      | %<VLF>pu
      | %<angleLF>deg.
      | %<Name>
  bus248 : powerlib/Measurements/Load Flow Bus  LConnTagsString=a  ID=bus248  Vbase=150000  Vref=1  Vangle=0  VLF=1  angleLF=0
      settings: AttributesFormatString=|
      | %<ID>
      | %<Vbase>V
      | %<VLF>pu
      | %<angleLF>deg.
      | %<Name>
  bus249 : powerlib/Measurements/Load Flow Bus  LConnTagsString=a  ID=bus249  Vbase=150000  Vref=1  Vangle=0  VLF=1  angleLF=0
      settings: AttributesFormatString=|
      | %<ID>
      | %<Vbase>V
      | %<VLF>pu
      | %<angleLF>deg.
      | %<Name>
  bus25 : powerlib/Measurements/Load Flow Bus  LConnTagsString=a  ID=bus25  Vbase=150000  Vref=1  Vangle=0  VLF=1  angleLF=0
      settings: AttributesFormatString=|
      | %<ID>
      | %<Vbase>V
      | %<VLF>pu
      | %<angleLF>deg.
      | %<Name>
  bus250 : powerlib/Measurements/Load Flow Bus  LConnTagsString=a  ID=bus250  Vbase=400000  Vref=1  Vangle=0  VLF=1  angleLF=0
      settings: AttributesFormatString=|
      | %<ID>
      | %<Vbase>V
      | %<VLF>pu
      | %<angleLF>deg.
      | %<Name>
  bus251 : powerlib/Measurements/Load Flow Bus  LConnTagsString=a  ID=bus251  Vbase=400000  Vref=1  Vangle=0  VLF=1  angleLF=0
      settings: AttributesFormatString=|
      | %<ID>
      | %<Vbase>V
      | %<VLF>pu
      | %<angleLF>deg.
      | %<Name>
  bus252 : powerlib/Measurements/Load Flow Bus  LConnTagsString=a  ID=bus252  Vbase=400000  Vref=1  Vangle=0  VLF=1  angleLF=0
      settings: AttributesFormatString=|
      | %<ID>
      | %<Vbase>V
      | %<VLF>pu
      | %<angleLF>deg.
      | %<Name>
  bus253 : powerlib/Measurements/Load Flow Bus  LConnTagsString=a  ID=bus253  Vbase=400000  Vref=1  Vangle=0  VLF=1  angleLF=0
      settings: AttributesFormatString=|
      | %<ID>
      | %<Vbase>V
      | %<VLF>pu
      | %<angleLF>deg.
      | %<Name>
  bus254 : powerlib/Measurements/Load Flow Bus  LConnTagsString=a  ID=bus254  Vbase=400000  Vref=1  Vangle=0  VLF=1  angleLF=0
      settings: AttributesFormatString=|
      | %<ID>
      | %<Vbase>V
      | %<VLF>pu
      | %<angleLF>deg.
      | %<Name>
  bus255 : powerlib/Measurements/Load Flow Bus  LConnTagsString=a  ID=bus255  Vbase=400000  Vref=1  Vangle=0  VLF=1  angleLF=0
      settings: AttributesFormatString=|
      | %<ID>
      | %<Vbase>V
      | %<VLF>pu
      | %<angleLF>deg.
      | %<Name>
  bus256 : powerlib/Measurements/Load Flow Bus  LConnTagsString=a  ID=bus256  Vbase=400000  Vref=1  Vangle=0  VLF=1  angleLF=0
      settings: AttributesFormatString=|
      | %<ID>
      | %<Vbase>V
      | %<VLF>pu
      | %<angleLF>deg.
      | %<Name>
  bus257 : powerlib/Measurements/Load Flow Bus  LConnTagsString=a  ID=bus257  Vbase=400000  Vref=1  Vangle=0  VLF=1  angleLF=0
      settings: AttributesFormatString=|
      | %<ID>
      | %<Vbase>V
      | %<VLF>pu
      | %<angleLF>deg.
      | %<Name>
  bus258 : powerlib/Measurements/Load Flow Bus  LConnTagsString=a  ID=bus258  Vbase=400000  Vref=1  Vangle=0  VLF=1  angleLF=0
      settings: AttributesFormatString=|
      | %<ID>
      | %<Vbase>V
      | %<VLF>pu
      | %<angleLF>deg.
      | %<Name>
  bus259 : powerlib/Measurements/Load Flow Bus  LConnTagsString=a  ID=bus259  Vbase=400000  Vref=1  Vangle=0  VLF=1  angleLF=0
      settings: AttributesFormatString=|
      | %<ID>
      | %<Vbase>V
      | %<VLF>pu
      | %<angleLF>deg.
      | %<Name>
  bus26 : powerlib/Measurements/Load Flow Bus  LConnTagsString=a  ID=bus26  Vbase=150000  Vref=1  Vangle=0  VLF=1  angleLF=0
      settings: AttributesFormatString=|
      | %<ID>
      | %<Vbase>V
      | %<VLF>pu
      | %<angleLF>deg.
      | %<Name>
  bus260 : powerlib/Measurements/Load Flow Bus  LConnTagsString=a  ID=bus260  Vbase=400000  Vref=1  Vangle=0  VLF=1  angleLF=0
      settings: AttributesFormatString=|
      | %<ID>
      | %<Vbase>V
      | %<VLF>pu
      | %<angleLF>deg.
      | %<Name>
  bus27 : powerlib/Measurements/Load Flow Bus  LConnTagsString=a  ID=bus27  Vbase=150000  Vref=1  Vangle=0  VLF=1  angleLF=0
      settings: AttributesFormatString=|
      | %<ID>
      | %<Vbase>V
      | %<VLF>pu
      | %<angleLF>deg.
      | %<Name>
  bus28 : powerlib/Measurements/Load Flow Bus  LConnTagsString=a  ID=bus28  Vbase=150000  Vref=1  Vangle=0  VLF=1  angleLF=0
      settings: AttributesFormatString=|
      | %<ID>
      | %<Vbase>V
      | %<VLF>pu
      | %<angleLF>deg.
      | %<Name>
  bus29 : powerlib/Measurements/Load Flow Bus  LConnTagsString=a  ID=bus29  Vbase=150000  Vref=1  Vangle=0  VLF=1  angleLF=0
      settings: AttributesFormatString=|
      | %<ID>
      | %<Vbase>V
      | %<VLF>pu
      | %<angleLF>deg.
      | %<Name>
  bus3 : powerlib/Measurements/Load Flow Bus  LConnTagsString=a  ID=bus3  Vbase=150000  Vref=1  Vangle=0  VLF=1  angleLF=0
      settings: AttributesFormatString=|
      | %<ID>
      | %<Vbase>V
      | %<VLF>pu
      | %<angleLF>deg.
      | %<Name>
  bus30 : powerlib/Measurements/Load Flow Bus  LConnTagsString=a  ID=bus30  Vbase=150000  Vref=1  Vangle=0  VLF=1  angleLF=0
      settings: AttributesFormatString=|
      | %<ID>
      | %<Vbase>V
      | %<VLF>pu
      | %<angleLF>deg.
      | %<Name>
  bus31 : powerlib/Measurements/Load Flow Bus  LConnTagsString=a  ID=bus31  Vbase=150000  Vref=1  Vangle=0  VLF=1  angleLF=0
      settings: AttributesFormatString=|
      | %<ID>
      | %<Vbase>V
      | %<VLF>pu
      | %<angleLF>deg.
      | %<Name>
  bus32 : powerlib/Measurements/Load Flow Bus  LConnTagsString=a  ID=bus32  Vbase=150000  Vref=1  Vangle=0  VLF=1  angleLF=0
      settings: AttributesFormatString=|
      | %<ID>
      | %<Vbase>V
      | %<VLF>pu
      | %<angleLF>deg.
      | %<Name>
  bus33 : powerlib/Measurements/Load Flow Bus  LConnTagsString=a  ID=bus33  Vbase=150000  Vref=1  Vangle=0  VLF=1  angleLF=0
      settings: AttributesFormatString=|
      | %<ID>
      | %<Vbase>V
      | %<VLF>pu
      | %<angleLF>deg.
      | %<Name>
  bus34 : powerlib/Measurements/Load Flow Bus  LConnTagsString=a  ID=bus34  Vbase=150000  Vref=1  Vangle=0  VLF=1  angleLF=0
      settings: AttributesFormatString=|
      | %<ID>
      | %<Vbase>V
      | %<VLF>pu
      | %<angleLF>deg.
      | %<Name>
  bus35 : powerlib/Measurements/Load Flow Bus  LConnTagsString=a  ID=bus35  Vbase=150000  Vref=1  Vangle=0  VLF=1  angleLF=0
      settings: AttributesFormatString=|
      | %<ID>
      | %<Vbase>V
      | %<VLF>pu
      | %<angleLF>deg.
      | %<Name>
  bus36 : powerlib/Measurements/Load Flow Bus  LConnTagsString=a  ID=bus36  Vbase=150000  Vref=1  Vangle=0  VLF=1  angleLF=0
      settings: AttributesFormatString=|
      | %<ID>
      | %<Vbase>V
      | %<VLF>pu
      | %<angleLF>deg.
      | %<Name>
  bus37 : powerlib/Measurements/Load Flow Bus  LConnTagsString=a  ID=bus37  Vbase=150000  Vref=1  Vangle=0  VLF=1  angleLF=0
      settings: AttributesFormatString=|
      | %<ID>
      | %<Vbase>V
      | %<VLF>pu
      | %<angleLF>deg.
      | %<Name>
  bus38 : powerlib/Measurements/Load Flow Bus  LConnTagsString=a  ID=bus38  Vbase=150000  Vref=1  Vangle=0  VLF=1  angleLF=0
      settings: AttributesFormatString=|
      | %<ID>
      | %<Vbase>V
      | %<VLF>pu
      | %<angleLF>deg.
      | %<Name>
  bus39 : powerlib/Measurements/Load Flow Bus  LConnTagsString=a  ID=bus39  Vbase=150000  Vref=1  Vangle=0  VLF=1  angleLF=0
      settings: AttributesFormatString=|
      | %<ID>
      | %<Vbase>V
      | %<VLF>pu
      | %<angleLF>deg.
      | %<Name>
  bus4 : powerlib/Measurements/Load Flow Bus  LConnTagsString=a  ID=bus4  Vbase=150000  Vref=1  Vangle=0  VLF=1  angleLF=0
      settings: AttributesFormatString=|
      | %<ID>
      | %<Vbase>V
      | %<VLF>pu
      | %<angleLF>deg.
      | %<Name>
  bus40 : powerlib/Measurements/Load Flow Bus  LConnTagsString=a  ID=bus40  Vbase=150000  Vref=1  Vangle=0  VLF=1  angleLF=0
      settings: AttributesFormatString=|
      | %<ID>
      | %<Vbase>V
      | %<VLF>pu
      | %<angleLF>deg.
      | %<Name>
  bus41 : powerlib/Measurements/Load Flow Bus  LConnTagsString=a  ID=bus41  Vbase=150000  Vref=1  Vangle=0  VLF=1  angleLF=0
      settings: AttributesFormatString=|
      | %<ID>
      | %<Vbase>V
      | %<VLF>pu
      | %<angleLF>deg.
      | %<Name>
  bus42 : powerlib/Measurements/Load Flow Bus  LConnTagsString=a  ID=bus42  Vbase=150000  Vref=1  Vangle=0  VLF=1  angleLF=0
      settings: AttributesFormatString=|
      | %<ID>
      | %<Vbase>V
      | %<VLF>pu
      | %<angleLF>deg.
      | %<Name>
  bus43 : powerlib/Measurements/Load Flow Bus  LConnTagsString=a  ID=bus43  Vbase=150000  Vref=1  Vangle=0  VLF=1  angleLF=0
      settings: AttributesFormatString=|
      | %<ID>
      | %<Vbase>V
      | %<VLF>pu
      | %<angleLF>deg.
      | %<Name>
  bus44 : powerlib/Measurements/Load Flow Bus  LConnTagsString=a  ID=bus44  Vbase=150000  Vref=1  Vangle=0  VLF=1  angleLF=0
      settings: AttributesFormatString=|
      | %<ID>
      | %<Vbase>V
      | %<VLF>pu
      | %<angleLF>deg.
      | %<Name>
  bus45 : powerlib/Measurements/Load Flow Bus  LConnTagsString=a  ID=bus45  Vbase=150000  Vref=1  Vangle=0  VLF=1  angleLF=0
      settings: AttributesFormatString=|
      | %<ID>
      | %<Vbase>V
      | %<VLF>pu
      | %<angleLF>deg.
      | %<Name>
  bus46 : powerlib/Measurements/Load Flow Bus  LConnTagsString=a  ID=bus46  Vbase=150000  Vref=1  Vangle=0  VLF=1  angleLF=0
      settings: AttributesFormatString=|
      | %<ID>
      | %<Vbase>V
      | %<VLF>pu
      | %<angleLF>deg.
      | %<Name>
  bus47 : powerlib/Measurements/Load Flow Bus  LConnTagsString=a  ID=bus47  Vbase=150000  Vref=1  Vangle=0  VLF=1  angleLF=0
      settings: AttributesFormatString=|
      | %<ID>
      | %<Vbase>V
      | %<VLF>pu
      | %<angleLF>deg.
      | %<Name>
  bus48 : powerlib/Measurements/Load Flow Bus  LConnTagsString=a  ID=bus48  Vbase=150000  Vref=1  Vangle=0  VLF=1  angleLF=0
      settings: AttributesFormatString=|
      | %<ID>
      | %<Vbase>V
      | %<VLF>pu
      | %<angleLF>deg.
      | %<Name>
  bus49 : powerlib/Measurements/Load Flow Bus  LConnTagsString=a  ID=bus49  Vbase=150000  Vref=1  Vangle=0  VLF=1  angleLF=0
      settings: AttributesFormatString=|
      | %<ID>
      | %<Vbase>V
      | %<VLF>pu
      | %<angleLF>deg.
      | %<Name>
  bus5 : powerlib/Measurements/Load Flow Bus  LConnTagsString=a  ID=bus5  Vbase=150000  Vref=1  Vangle=0  VLF=1  angleLF=0
      settings: AttributesFormatString=|
      | %<ID>
      | %<Vbase>V
      | %<VLF>pu
      | %<angleLF>deg.
      | %<Name>
  bus50 : powerlib/Measurements/Load Flow Bus  LConnTagsString=a  ID=bus50  Vbase=150000  Vref=1  Vangle=0  VLF=1  angleLF=0
      settings: AttributesFormatString=|
      | %<ID>
      | %<Vbase>V
      | %<VLF>pu
      | %<angleLF>deg.
      | %<Name>
  bus51 : powerlib/Measurements/Load Flow Bus  LConnTagsString=a  ID=bus51  Vbase=150000  Vref=1  Vangle=0  VLF=1  angleLF=0
      settings: AttributesFormatString=|
      | %<ID>
      | %<Vbase>V
      | %<VLF>pu
      | %<angleLF>deg.
      | %<Name>
  bus52 : powerlib/Measurements/Load Flow Bus  LConnTagsString=a  ID=bus52  Vbase=150000  Vref=1  Vangle=0  VLF=1  angleLF=0
      settings: AttributesFormatString=|
      | %<ID>
      | %<Vbase>V
      | %<VLF>pu
      | %<angleLF>deg.
      | %<Name>
  bus53 : powerlib/Measurements/Load Flow Bus  LConnTagsString=a  ID=bus53  Vbase=150000  Vref=1  Vangle=0  VLF=1  angleLF=0
      settings: AttributesFormatString=|
      | %<ID>
      | %<Vbase>V
      | %<VLF>pu
      | %<angleLF>deg.
      | %<Name>
  bus54 : powerlib/Measurements/Load Flow Bus  LConnTagsString=a  ID=bus54  Vbase=150000  Vref=1  Vangle=0  VLF=1  angleLF=0
      settings: AttributesFormatString=|
      | %<ID>
      | %<Vbase>V
      | %<VLF>pu
      | %<angleLF>deg.
      | %<Name>
  bus55 : powerlib/Measurements/Load Flow Bus  LConnTagsString=a  ID=bus55  Vbase=150000  Vref=1  Vangle=0  VLF=1  angleLF=0
      settings: AttributesFormatString=|
      | %<ID>
      | %<Vbase>V
      | %<VLF>pu
      | %<angleLF>deg.
      | %<Name>
  bus56 : powerlib/Measurements/Load Flow Bus  LConnTagsString=a  ID=bus56  Vbase=150000  Vref=1  Vangle=0  VLF=1  angleLF=0
      settings: AttributesFormatString=|
      | %<ID>
      | %<Vbase>V
      | %<VLF>pu
      | %<angleLF>deg.
      | %<Name>
  bus57 : powerlib/Measurements/Load Flow Bus  LConnTagsString=a  ID=bus57  Vbase=150000  Vref=1  Vangle=0  VLF=1  angleLF=0
      settings: AttributesFormatString=|
      | %<ID>
      | %<Vbase>V
      | %<VLF>pu
      | %<angleLF>deg.
      | %<Name>
  bus58 : powerlib/Measurements/Load Flow Bus  LConnTagsString=a  ID=bus58  Vbase=150000  Vref=1  Vangle=0  VLF=1  angleLF=0
      settings: AttributesFormatString=|
      | %<ID>
      | %<Vbase>V
      | %<VLF>pu
      | %<angleLF>deg.
      | %<Name>
  bus59 : powerlib/Measurements/Load Flow Bus  LConnTagsString=a  ID=bus59  Vbase=150000  Vref=1  Vangle=0  VLF=1  angleLF=0
      settings: AttributesFormatString=|
      | %<ID>
      | %<Vbase>V
      | %<VLF>pu
      | %<angleLF>deg.
      | %<Name>
  bus6 : powerlib/Measurements/Load Flow Bus  LConnTagsString=a  ID=bus6  Vbase=150000  Vref=1  Vangle=0  VLF=1  angleLF=0
      settings: AttributesFormatString=|
      | %<ID>
      | %<Vbase>V
      | %<VLF>pu
      | %<angleLF>deg.
      | %<Name>
  bus60 : powerlib/Measurements/Load Flow Bus  LConnTagsString=a  ID=bus60  Vbase=150000  Vref=1  Vangle=0  VLF=1  angleLF=0
      settings: AttributesFormatString=|
      | %<ID>
      | %<Vbase>V
      | %<VLF>pu
      | %<angleLF>deg.
      | %<Name>
  bus61 : powerlib/Measurements/Load Flow Bus  LConnTagsString=a  ID=bus61  Vbase=150000  Vref=1  Vangle=0  VLF=1  angleLF=0
      settings: AttributesFormatString=|
      | %<ID>
      | %<Vbase>V
      | %<VLF>pu
      | %<angleLF>deg.
      | %<Name>
  bus62 : powerlib/Measurements/Load Flow Bus  LConnTagsString=a  ID=bus62  Vbase=150000  Vref=1  Vangle=0  VLF=1  angleLF=0
      settings: AttributesFormatString=|
      | %<ID>
      | %<Vbase>V
      | %<VLF>pu
      | %<angleLF>deg.
      | %<Name>
  bus63 : powerlib/Measurements/Load Flow Bus  LConnTagsString=a  ID=bus63  Vbase=150000  Vref=1  Vangle=0  VLF=1  angleLF=0
      settings: AttributesFormatString=|
      | %<ID>
      | %<Vbase>V
      | %<VLF>pu
      | %<angleLF>deg.
      | %<Name>
  bus64 : powerlib/Measurements/Load Flow Bus  LConnTagsString=a  ID=bus64  Vbase=150000  Vref=1  Vangle=0  VLF=1  angleLF=0
      settings: AttributesFormatString=|
      | %<ID>
      | %<Vbase>V
      | %<VLF>pu
      | %<angleLF>deg.
      | %<Name>
  bus65 : powerlib/Measurements/Load Flow Bus  LConnTagsString=a  ID=bus65  Vbase=150000  Vref=1  Vangle=0  VLF=1  angleLF=0
      settings: AttributesFormatString=|
      | %<ID>
      | %<Vbase>V
      | %<VLF>pu
      | %<angleLF>deg.
      | %<Name>
  bus66 : powerlib/Measurements/Load Flow Bus  LConnTagsString=a  ID=bus66  Vbase=150000  Vref=1  Vangle=0  VLF=1  angleLF=0
      settings: AttributesFormatString=|
      | %<ID>
      | %<Vbase>V
      | %<VLF>pu
      | %<angleLF>deg.
      | %<Name>
  bus67 : powerlib/Measurements/Load Flow Bus  LConnTagsString=a  ID=bus67  Vbase=150000  Vref=1  Vangle=0  VLF=1  angleLF=0
      settings: AttributesFormatString=|
      | %<ID>
      | %<Vbase>V
      | %<VLF>pu
      | %<angleLF>deg.
      | %<Name>
  bus68 : powerlib/Measurements/Load Flow Bus  LConnTagsString=a  ID=bus68  Vbase=150000  Vref=1  Vangle=0  VLF=1  angleLF=0
      settings: AttributesFormatString=|
      | %<ID>
      | %<Vbase>V
      | %<VLF>pu
      | %<angleLF>deg.
      | %<Name>
  bus69 : powerlib/Measurements/Load Flow Bus  LConnTagsString=a  ID=bus69  Vbase=150000  Vref=1  Vangle=0  VLF=1  angleLF=0
      settings: AttributesFormatString=|
      | %<ID>
      | %<Vbase>V
      | %<VLF>pu
      | %<angleLF>deg.
      | %<Name>
  bus7 : powerlib/Measurements/Load Flow Bus  LConnTagsString=a  ID=bus7  Vbase=150000  Vref=1  Vangle=0  VLF=1  angleLF=0
      settings: AttributesFormatString=|
      | %<ID>
      | %<Vbase>V
      | %<VLF>pu
      | %<angleLF>deg.
      | %<Name>
  bus70 : powerlib/Measurements/Load Flow Bus  LConnTagsString=a  ID=bus70  Vbase=150000  Vref=1  Vangle=0  VLF=1  angleLF=0
      settings: AttributesFormatString=|
      | %<ID>
      | %<Vbase>V
      | %<VLF>pu
      | %<angleLF>deg.
      | %<Name>
  bus71 : powerlib/Measurements/Load Flow Bus  LConnTagsString=a  ID=bus71  Vbase=150000  Vref=1  Vangle=0  VLF=1  angleLF=0
      settings: AttributesFormatString=|
      | %<ID>
      | %<Vbase>V
      | %<VLF>pu
      | %<angleLF>deg.
      | %<Name>
  bus72 : powerlib/Measurements/Load Flow Bus  LConnTagsString=a  ID=bus72  Vbase=150000  Vref=1  Vangle=0  VLF=1  angleLF=0
      settings: AttributesFormatString=|
      | %<ID>
      | %<Vbase>V
      | %<VLF>pu
      | %<angleLF>deg.
      | %<Name>
  bus73 : powerlib/Measurements/Load Flow Bus  LConnTagsString=a  ID=bus73  Vbase=150000  Vref=1  Vangle=0  VLF=1  angleLF=0
      settings: AttributesFormatString=|
      | %<ID>
      | %<Vbase>V
      | %<VLF>pu
      | %<angleLF>deg.
      | %<Name>
  bus74 : powerlib/Measurements/Load Flow Bus  LConnTagsString=a  ID=bus74  Vbase=150000  Vref=1  Vangle=0  VLF=1  angleLF=0
      settings: AttributesFormatString=|
      | %<ID>
      | %<Vbase>V
      | %<VLF>pu
      | %<angleLF>deg.
      | %<Name>
  bus75 : powerlib/Measurements/Load Flow Bus  LConnTagsString=a  ID=bus75  Vbase=150000  Vref=1  Vangle=0  VLF=1  angleLF=0
      settings: AttributesFormatString=|
      | %<ID>
      | %<Vbase>V
      | %<VLF>pu
      | %<angleLF>deg.
      | %<Name>
  bus76 : powerlib/Measurements/Load Flow Bus  LConnTagsString=a  ID=bus76  Vbase=150000  Vref=1  Vangle=0  VLF=1  angleLF=0
      settings: AttributesFormatString=|
      | %<ID>
      | %<Vbase>V
      | %<VLF>pu
      | %<angleLF>deg.
      | %<Name>
  bus77 : powerlib/Measurements/Load Flow Bus  LConnTagsString=a  ID=bus77  Vbase=150000  Vref=1  Vangle=0  VLF=1  angleLF=0
      settings: AttributesFormatString=|
      | %<ID>
      | %<Vbase>V
      | %<VLF>pu
      | %<angleLF>deg.
      | %<Name>
  bus78 : powerlib/Measurements/Load Flow Bus  LConnTagsString=a  ID=bus78  Vbase=150000  Vref=1  Vangle=0  VLF=1  angleLF=0
      settings: AttributesFormatString=|
      | %<ID>
      | %<Vbase>V
      | %<VLF>pu
      | %<angleLF>deg.
      | %<Name>
  bus79 : powerlib/Measurements/Load Flow Bus  LConnTagsString=a  ID=bus79  Vbase=150000  Vref=1  Vangle=0  VLF=1  angleLF=0
      settings: AttributesFormatString=|
      | %<ID>
      | %<Vbase>V
      | %<VLF>pu
      | %<angleLF>deg.
      | %<Name>
  bus8 : powerlib/Measurements/Load Flow Bus  LConnTagsString=a  ID=bus8  Vbase=150000  Vref=1  Vangle=0  VLF=1  angleLF=0
      settings: AttributesFormatString=|
      | %<ID>
      | %<Vbase>V
      | %<VLF>pu
      | %<angleLF>deg.
      | %<Name>
  bus80 : powerlib/Measurements/Load Flow Bus  LConnTagsString=a  ID=bus80  Vbase=150000  Vref=1  Vangle=0  VLF=1  angleLF=0
      settings: AttributesFormatString=|
      | %<ID>
      | %<Vbase>V
      | %<VLF>pu
      | %<angleLF>deg.
      | %<Name>
  bus81 : powerlib/Measurements/Load Flow Bus  LConnTagsString=a  ID=bus81  Vbase=150000  Vref=1  Vangle=0  VLF=1  angleLF=0
      settings: AttributesFormatString=|
      | %<ID>
      | %<Vbase>V
      | %<VLF>pu
      | %<angleLF>deg.
      | %<Name>
  bus82 : powerlib/Measurements/Load Flow Bus  LConnTagsString=a  ID=bus82  Vbase=150000  Vref=1  Vangle=0  VLF=1  angleLF=0
      settings: AttributesFormatString=|
      | %<ID>
      | %<Vbase>V
      | %<VLF>pu
      | %<angleLF>deg.
      | %<Name>
  bus83 : powerlib/Measurements/Load Flow Bus  LConnTagsString=a  ID=bus83  Vbase=150000  Vref=1  Vangle=0  VLF=1  angleLF=0
      settings: AttributesFormatString=|
      | %<ID>
      | %<Vbase>V
      | %<VLF>pu
      | %<angleLF>deg.
      | %<Name>
  bus84 : powerlib/Measurements/Load Flow Bus  LConnTagsString=a  ID=bus84  Vbase=150000  Vref=1  Vangle=0  VLF=1  angleLF=0
      settings: AttributesFormatString=|
      | %<ID>
      | %<Vbase>V
      | %<VLF>pu
      | %<angleLF>deg.
      | %<Name>
  bus85 : powerlib/Measurements/Load Flow Bus  LConnTagsString=a  ID=bus85  Vbase=150000  Vref=1  Vangle=0  VLF=1  angleLF=0
      settings: AttributesFormatString=|
      | %<ID>
      | %<Vbase>V
      | %<VLF>pu
      | %<angleLF>deg.
      | %<Name>
  bus86 : powerlib/Measurements/Load Flow Bus  LConnTagsString=a  ID=bus86  Vbase=150000  Vref=1  Vangle=0  VLF=1  angleLF=0
      settings: AttributesFormatString=|
      | %<ID>
      | %<Vbase>V
      | %<VLF>pu
      | %<angleLF>deg.
      | %<Name>
  bus87 : powerlib/Measurements/Load Flow Bus  LConnTagsString=a  ID=bus87  Vbase=150000  Vref=1  Vangle=0  VLF=1  angleLF=0
      settings: AttributesFormatString=|
      | %<ID>
      | %<Vbase>V
      | %<VLF>pu
      | %<angleLF>deg.
      | %<Name>
  bus88 : powerlib/Measurements/Load Flow Bus  LConnTagsString=a  ID=bus88  Vbase=150000  Vref=1  Vangle=0  VLF=1  angleLF=0
      settings: AttributesFormatString=|
      | %<ID>
      | %<Vbase>V
      | %<VLF>pu
      | %<angleLF>deg.
      | %<Name>
  bus89 : powerlib/Measurements/Load Flow Bus  LConnTagsString=a  ID=bus89  Vbase=150000  Vref=1  Vangle=0  VLF=1  angleLF=0
      settings: AttributesFormatString=|
      | %<ID>
      | %<Vbase>V
      | %<VLF>pu
      | %<angleLF>deg.
      | %<Name>
  bus9 : powerlib/Measurements/Load Flow Bus  LConnTagsString=a  ID=bus9  Vbase=150000  Vref=1  Vangle=0  VLF=1  angleLF=0
      settings: AttributesFormatString=|
      | %<ID>
      | %<Vbase>V
      | %<VLF>pu
      | %<angleLF>deg.
      | %<Name>
  bus90 : powerlib/Measurements/Load Flow Bus  LConnTagsString=a  ID=bus90  Vbase=150000  Vref=1  Vangle=0  VLF=1  angleLF=0
      settings: AttributesFormatString=|
      | %<ID>
      | %<Vbase>V
      | %<VLF>pu
      | %<angleLF>deg.
      | %<Name>
  bus91 : powerlib/Measurements/Load Flow Bus  LConnTagsString=a  ID=bus91  Vbase=150000  Vref=1  Vangle=0  VLF=1  angleLF=0
      settings: AttributesFormatString=|
      | %<ID>
      | %<Vbase>V
      | %<VLF>pu
      | %<angleLF>deg.
      | %<Name>
  bus92 : powerlib/Measurements/Load Flow Bus  LConnTagsString=a  ID=bus92  Vbase=150000  Vref=1  Vangle=0  VLF=1  angleLF=0
      settings: AttributesFormatString=|
      | %<ID>
      | %<Vbase>V
      | %<VLF>pu
      | %<angleLF>deg.
      | %<Name>
  bus93 : powerlib/Measurements/Load Flow Bus  LConnTagsString=a  ID=bus93  Vbase=150000  Vref=1  Vangle=0  VLF=1  angleLF=0
      settings: AttributesFormatString=|
      | %<ID>
      | %<Vbase>V
      | %<VLF>pu
      | %<angleLF>deg.
      | %<Name>
  bus94 : powerlib/Measurements/Load Flow Bus  LConnTagsString=a  ID=bus94  Vbase=150000  Vref=1  Vangle=0  VLF=1  angleLF=0
      settings: AttributesFormatString=|
      | %<ID>
      | %<Vbase>V
      | %<VLF>pu
      | %<angleLF>deg.
      | %<Name>
  bus95 : powerlib/Measurements/Load Flow Bus  LConnTagsString=a  ID=bus95  Vbase=150000  Vref=1  Vangle=0  VLF=1  angleLF=0
      settings: AttributesFormatString=|
      | %<ID>
      | %<Vbase>V
      | %<VLF>pu
      | %<angleLF>deg.
      | %<Name>
  bus96 : powerlib/Measurements/Load Flow Bus  LConnTagsString=a  ID=bus96  Vbase=150000  Vref=1  Vangle=0  VLF=1  angleLF=0
      settings: AttributesFormatString=|
      | %<ID>
      | %<Vbase>V
      | %<VLF>pu
      | %<angleLF>deg.
      | %<Name>
  bus97 : powerlib/Measurements/Load Flow Bus  LConnTagsString=a  ID=bus97  Vbase=150000  Vref=1  Vangle=0  VLF=1  angleLF=0
      settings: AttributesFormatString=|
      | %<ID>
      | %<Vbase>V
      | %<VLF>pu
      | %<angleLF>deg.
      | %<Name>
  bus98 : powerlib/Measurements/Load Flow Bus  LConnTagsString=a  ID=bus98  Vbase=150000  Vref=1  Vangle=0  VLF=1  angleLF=0
      settings: AttributesFormatString=|
      | %<ID>
      | %<Vbase>V
      | %<VLF>pu
      | %<angleLF>deg.
      | %<Name>
  bus99 : powerlib/Measurements/Load Flow Bus  LConnTagsString=a  ID=bus99  Vbase=150000  Vref=1  Vangle=0  VLF=1  angleLF=0
      settings: AttributesFormatString=|
      | %<ID>
      | %<Vbase>V
      | %<VLF>pu
      | %<angleLF>deg.
      | %<Name>
  powergui : powerlib/powergui  Priority=1  SimulationMode=Continuous  SolverType=Tustin  SampleTime=50e-6  frequency=60  SPID=off  DisableSnubberDevices=off  DisableRonSwitches=off  DisableVfSwitches=off  SwTol=0  Interpol=off  DisplayEquations=off  Ts=0  methode=off  frequencyindice=60  Pbase=100e6  ErrMax=1e-4  Iterations=50  UnitsV=kV  UnitsW=MW  FunctionMessages=off  echomessages=off  HookPort=off  EnableUseOfTLC=off  x0status=blocks  RestoreLinks=warning  ResistiveCurrentMeasurement=off  Frange=[0:2:500]  Ylog=off  Xlog=on  ShowGrid=off  save=off  variable=ZData  structure=0  ZoomFFT=off  StartTime=0.0  cycles=1  DisplayStyle=1  fundamental=60  FreqAxis=off  MaxFrequency=1000  frequencyindicesteady=1  RmsSteady=1  display=off
  Γ_Μ__ΚΥΤ_Διστόμου___ΚΥΤ_Κουμουνδούρου_CN_51408420_150000_CN_85518393_150000 : powerlib/Elements/Distributed Parameters Line  Phases=3  Frequency=60  Resistance=[0.01273 0.3864]  Inductance="[0.9337e-3  4.1264e-3]"  Capacitance=[12.74e-9 7.751e-9]  Length=78.6102  x1=[0 0 0 0; 0.0001244 0 0 0; 0.0002488 0 0 0; 0.0003733 0 0 0; 0.0004977 0 0 0; 0.0006221 0 0 0]  x2=[0 0 0 0; 0.0001244 0 0 0; 0.0002488 0 0 0; 0.0003733 0 0 0; 0.0004977 0 0 0; 0.0006221 0 0 0]  x3=[0 0 0 0; 0.0001244 0 0 0; 0.0002488 0 0 0; 0.0003733 0 0 0; 0.0004977 0 0 0; 0.0006221 0 0 0]  x4=[0 0 0 0; 0.0001244 0 0 0; 0.0002488 0 0 0; 0.0003733 0 0 0; 0.0004977 0 0 0; 0.0006221 0 0 0]  x5=0  V1=ones(3,3)  V2=ones(3,3)  I1=ones(3,3)  I2=ones(3,3)  nHarmo=1  Measurements=None
  Γραμμή_400_kV_ΚΥΤ_Αράχθου___ΚΥΤ_Αχελώου_CN_105184051_400000_CN_140248148_400000 : powerlib/Elements/Distributed Parameters Line  Phases=3  Frequency=60  Resistance=[0.01273 0.3864]  Inductance="[0.9337e-3  4.1264e-3]"  Capacitance=[12.74e-9 7.751e-9]  Length=72.25  x1=[0 0 0 0; 0.0001244 0 0 0; 0.0002488 0 0 0; 0.0003733 0 0 0; 0.0004977 0 0 0; 0.0006221 0 0 0]  x2=[0 0 0 0; 0.0001244 0 0 0; 0.0002488 0 0 0; 0.0003733 0 0 0; 0.0004977 0 0 0; 0.0006221 0 0 0]  x3=[0 0 0 0; 0.0001244 0 0 0; 0.0002488 0 0 0; 0.0003733 0 0 0; 0.0004977 0 0 0; 0.0006221 0 0 0]  x4=[0 0 0 0; 0.0001244 0 0 0; 0.0002488 0 0 0; 0.0003733 0 0 0; 0.0004977 0 0 0; 0.0006221 0 0 0]  x5=0  V1=ones(3,3)  V2=ones(3,3)  I1=ones(3,3)  I2=ones(3,3)  nHarmo=1  Measurements=None
  Γραμμή_400_kV_ΚΥΤ_Αράχθου___ΚΥΤ_Τρικάλων_CN_149672244_400000_CN_140248148_400000 : powerlib/Elements/Distributed Parameters Line  Phases=3  Frequency=60  Resistance=[0.01273 0.3864]  Inductance="[0.9337e-3  4.1264e-3]"  Capacitance=[12.74e-9 7.751e-9]  Length=25.8995  x1=[0 0 0 0; 0.0001244 0 0 0; 0.0002488 0 0 0; 0.0003733 0 0 0; 0.0004977 0 0 0; 0.0006221 0 0 0]  x2=[0 0 0 0; 0.0001244 0 0 0; 0.0002488 0 0 0; 0.0003733 0 0 0; 0.0004977 0 0 0; 0.0006221 0 0 0]  x3=[0 0 0 0; 0.0001244 0 0 0; 0.0002488 0 0 0; 0.0003733 0 0 0; 0.0004977 0 0 0; 0.0006221 0 0 0]  x4=[0 0 0 0; 0.0001244 0 0 0; 0.0002488 0 0 0; 0.0003733 0 0 0; 0.0004977 0 0 0; 0.0006221 0 0 0]  x5=0  V1=ones(3,3)  V2=ones(3,3)  I1=ones(3,3)  I2=ones(3,3)  nHarmo=1  Measurements=None
  Γραμμή_400_kV_ΚΥΤ_Θεσσαλονίκης_–_ΚΥΤ_Φιλίππων_CN_55099563_400000_CN_302950604_400000 : powerlib/Elements/Distributed Parameters Line  Phases=3  Frequency=60  Resistance=[0.01273 0.3864]  Inductance="[0.9337e-3  4.1264e-3]"  Capacitance=[12.74e-9 7.751e-9]  Length=22.936  x1=[0 0 0 0; 0.0001244 0 0 0; 0.0002488 0 0 0; 0.0003733 0 0 0; 0.0004977 0 0 0; 0.0006221 0 0 0]  x2=[0 0 0 0; 0.0001244 0 0 0; 0.0002488 0 0 0; 0.0003733 0 0 0; 0.0004977 0 0 0; 0.0006221 0 0 0]  x3=[0 0 0 0; 0.0001244 0 0 0; 0.0002488 0 0 0; 0.0003733 0 0 0; 0.0004977 0 0 0; 0.0006221 0 0 0]  x4=[0 0 0 0; 0.0001244 0 0 0; 0.0002488 0 0 0; 0.0003733 0 0 0; 0.0004977 0 0 0; 0.0006221 0 0 0]  x5=0  V1=ones(3,3)  V2=ones(3,3)  I1=ones(3,3)  I2=ones(3,3)  nHarmo=1  Measurements=None
  Γραμμή_400_kV_ΚΥΤ_Φιλίππων_–_ΚΥΤ_Νέας_Σάντας_CN_140465679_400000_CN_141220249_400000 : powerlib/Elements/Distributed Parameters Line  Phases=3  Frequency=60  Resistance=[0.01273 0.3864]  Inductance="[0.9337e-3  4.1264e-3]"  Capacitance=[12.74e-9 7.751e-9]  Length=62.3583  x1=[0 0 0 0; 0.0001244 0 0 0; 0.0002488 0 0 0; 0.0003733 0 0 0; 0.0004977 0 0 0; 0.0006221 0 0 0]  x2=[0 0 0 0; 0.0001244 0 0 0; 0.0002488 0 0 0; 0.0003733 0 0 0; 0.0004977 0 0 0; 0.0006221 0 0 0]  x3=[0 0 0 0; 0.0001244 0 0 0; 0.0002488 0 0 0; 0.0003733 0 0 0; 0.0004977 0 0 0; 0.0006221 0 0 0]  x4=[0 0 0 0; 0.0001244 0 0 0; 0.0002488 0 0 0; 0.0003733 0 0 0; 0.0004977 0 0 0; 0.0006221 0 0 0]  x5=0  V1=ones(3,3)  V2=ones(3,3)  I1=ones(3,3)  I2=ones(3,3)  nHarmo=1  Measurements=None
  Пирин_CN_235044638_400000_CN_55099563_400000 : powerlib/Elements/Distributed Parameters Line  Phases=3  Frequency=60  Resistance=[0.01273 0.3864]  Inductance="[0.9337e-3  4.1264e-3]"  Capacitance=[12.74e-9 7.751e-9]  Length=99.6339  x1=[0 0 0 0; 0.0001244 0 0 0; 0.0002488 0 0 0; 0.0003733 0 0 0; 0.0004977 0 0 0; 0.0006221 0 0 0]  x2=[0 0 0 0; 0.0001244 0 0 0; 0.0002488 0 0 0; 0.0003733 0 0 0; 0.0004977 0 0 0; 0.0006221 0 0 0]  x3=[0 0 0 0; 0.0001244 0 0 0; 0.0002488 0 0 0; 0.0003733 0 0 0; 0.0004977 0 0 0; 0.0006221 0 0 0]  x4=[0 0 0 0; 0.0001244 0 0 0; 0.0002488 0 0 0; 0.0003733 0 0 0; 0.0004977 0 0 0; 0.0006221 0 0 0]  x5=0  V1=ones(3,3)  V2=ones(3,3)  I1=ones(3,3)  I2=ones(3,3)  nHarmo=1  Measurements=None
  connections:
  T_134685185__/LConn1 -- _CN_134685185_150000_CN_85612093_150000/LConn1
  T_134685185__/LConn2 -- _CN_134685185_150000_CN_85612093_150000/LConn2
  _CN_134685185_150000_CN_85612093_150000/LConn3 -- T_134685185__/LConn3 -- bus1/LConn1
  _CN_134685185_150000_CN_85612093_150000/RConn1 -- T_85612093__/RConn1 -- _CN_85612093_150000_CN_86466243_150000/LConn1 -- L_85612093/LConn1 -- _CN_85612093_150000_CN_134630651_150000/LConn1 -- _CN_85612093_150000_CN_93583004_150000/LConn1
  _CN_134685185_150000_CN_85612093_150000/RConn2 -- T_85612093__/RConn2 -- _CN_85612093_150000_CN_86466243_150000/LConn2 -- L_85612093/LConn2 -- _CN_85612093_150000_CN_134630651_150000/LConn2 -- _CN_85612093_150000_CN_93583004_150000/LConn2
  _CN_134685185_150000_CN_85612093_150000/RConn3 -- T_85612093__/RConn3 -- _CN_85612093_150000_CN_86466243_150000/LConn3 -- L_85612093/LConn3 -- bus2/LConn1 -- _CN_85612093_150000_CN_134630651_150000/LConn3 -- _CN_85612093_150000_CN_93583004_150000/LConn3
  _CN_93383685_150000_CN_135706289_150000/LConn1 -- T_93383685__/RConn1 -- _CN_93383685_150000_CN_15642023_150000/LConn1 -- L_93383685/LConn1
  _CN_93383685_150000_CN_135706289_150000/LConn2 -- T_93383685__/RConn2 -- _CN_93383685_150000_CN_15642023_150000/LConn2 -- L_93383685/LConn2
  _CN_93383685_150000_CN_135706289_150000/LConn3 -- T_93383685__/RConn3 -- _CN_93383685_150000_CN_15642023_150000/LConn3 -- L_93383685/LConn3 -- bus3/LConn1
  T_135706289__/LConn1 -- _CN_93383685_150000_CN_135706289_150000/RConn1
  T_135706289__/LConn2 -- _CN_93383685_150000_CN_135706289_150000/RConn2
  _CN_93383685_150000_CN_135706289_150000/RConn3 -- T_135706289__/LConn3 -- bus4/LConn1
  _CN_93383685_150000_CN_15642023_150000/RConn1 -- G_15642023_Ατμοηλεκτρικος_Σταθμος_Καρδίας/RConn1 -- _CN_252802673_150000_CN_15642023_150000/LConn1 -- _CN_93383685_400000_CN_15642023_150000/LConn1
  _CN_93383685_150000_CN_15642023_150000/RConn2 -- G_15642023_Ατμοηλεκτρικος_Σταθμος_Καρδίας/RConn2 -- _CN_252802673_150000_CN_15642023_150000/LConn2 -- _CN_93383685_400000_CN_15642023_150000/LConn2
  _CN_93383685_150000_CN_15642023_150000/RConn3 -- G_15642023_Ατμοηλεκτρικος_Σταθμος_Καρδίας/RConn3 -- _CN_252802673_150000_CN_15642023_150000/LConn3 -- _CN_93383685_400000_CN_15642023_150000/LConn3 -- bus5/LConn1
  T_96020492__/LConn1 -- _CN_96020492_150000_CN_96314289_150000/LConn1
  T_96020492__/LConn2 -- _CN_96020492_150000_CN_96314289_150000/LConn2
  _CN_96020492_150000_CN_96314289_150000/LConn3 -- T_96020492__/LConn3 -- bus6/LConn1
  _CN_96020492_150000_CN_96314289_150000/RConn1 -- T_96314289__/LConn1 -- _CN_96040696_150000_CN_96314289_150000/LConn1 -- _CN_96314286_150000_CN_96314289_150000/LConn1
  _CN_96020492_150000_CN_96314289_150000/RConn2 -- T_96314289__/LConn2 -- _CN_96040696_150000_CN_96314289_150000/LConn2 -- _CN_96314286_150000_CN_96314289_150000/LConn2
  _CN_96020492_150000_CN_96314289_150000/RConn3 -- T_96314289__/LConn3 -- _CN_96040696_150000_CN_96314289_150000/LConn3 -- _CN_96314286_150000_CN_96314289_150000/LConn3 -- bus7/LConn1
  _CN_140465679_150000_CN_140343651_150000/LConn1 -- T_140465679__Κέντρο_Υπερυψηλής_Τάσης_(ΚΥΤ)_Φιλίππων/RConn1 -- _CN_140465679_150000_CN_55099563_150000/LConn1 -- _CN_140465679_150000_CN_132381638_150000/LConn1 -- _CN_140465679_150000_CN_72180968_150000/LConn1 -- L_140465679/LConn1
  _CN_140465679_150000_CN_140343651_150000/LConn2 -- T_140465679__Κέντρο_Υπερυψηλής_Τάσης_(ΚΥΤ)_Φιλίππων/RConn2 -- _CN_140465679_150000_CN_55099563_150000/LConn2 -- _CN_140465679_150000_CN_132381638_150000/LConn2 -- _CN_140465679_150000_CN_72180968_150000/LConn2 -- L_140465679/LConn2
  _CN_140465679_150000_CN_140343651_150000/LConn3 -- T_140465679__Κέντρο_Υπερυψηλής_Τάσης_(ΚΥΤ)_Φιλίππων/RConn3 -- _CN_140465679_150000_CN_55099563_150000/LConn3 -- _CN_140465679_150000_CN_132381638_150000/LConn3 -- _CN_140465679_150000_CN_72180968_150000/LConn3 -- L_140465679/LConn3 -- bus8/LConn1
  T_140343651__/LConn1 -- _CN_140465679_150000_CN_140343651_150000/RConn1
  T_140343651__/LConn2 -- _CN_140465679_150000_CN_140343651_150000/RConn2
  _CN_140465679_150000_CN_140343651_150000/RConn3 -- T_140343651__/LConn3 -- bus9/LConn1
  _CN_140465679_150000_CN_55099563_150000/RConn1 -- T_55099563_400000;150000_Κέντρο_Υπερυψηλής_Τάσης_Θεσσαλονίκης_(ΚΥΤ_Ωραιοκάστρου)/RConn1 -- _CN_55099563_150000_CN_92508649_150000/LConn1 -- _CN_55099563_150000_CN_92508651_150000/LConn1 -- L_55099563/LConn1 -- _CN_141514344_150000_CN_55099563_150000/LConn1 -- _CN_55099563_150000_CN_159413454_150000/LConn1 -- _CN_279628389_150000_CN_55099563_150000/LConn1
  _CN_140465679_150000_CN_55099563_150000/RConn2 -- T_55099563_400000;150000_Κέντρο_Υπερυψηλής_Τάσης_Θεσσαλονίκης_(ΚΥΤ_Ωραιοκάστρου)/RConn2 -- _CN_55099563_150000_CN_92508649_150000/LConn2 -- _CN_55099563_150000_CN_92508651_150000/LConn2 -- L_55099563/LConn2 -- _CN_141514344_150000_CN_55099563_150000/LConn2 -- _CN_55099563_150000_CN_159413454_150000/LConn2 -- _CN_279628389_150000_CN_55099563_150000/LConn2
  _CN_140465679_150000_CN_55099563_150000/RConn3 -- T_55099563_400000;150000_Κέντρο_Υπερυψηλής_Τάσης_Θεσσαλονίκης_(ΚΥΤ_Ωραιοκάστρου)/RConn3 -- _CN_55099563_150000_CN_92508649_150000/LConn3 -- _CN_55099563_150000_CN_92508651_150000/LConn3 -- L_55099563/LConn3 -- bus10/LConn1 -- _CN_141514344_150000_CN_55099563_150000/LConn3 -- _CN_55099563_150000_CN_159413454_150000/LConn3 -- _CN_279628389_150000_CN_55099563_150000/LConn3
  T_132381638__/LConn1 -- _CN_140465679_150000_CN_132381638_150000/RConn1
  T_132381638__/LConn2 -- _CN_140465679_150000_CN_132381638_150000/RConn2
  _CN_140465679_150000_CN_132381638_150000/RConn3 -- T_132381638__/LConn3 -- bus11/LConn1
  T_72180968__/LConn1 -- _CN_140465679_150000_CN_72180968_150000/RConn1
  T_72180968__/LConn2 -- _CN_140465679_150000_CN_72180968_150000/RConn2
  _CN_140465679_150000_CN_72180968_150000/RConn3 -- T_72180968__/LConn3 -- bus12/LConn1
  _CN_92611161_150000_CN_92611154_150000/LConn1 -- T_92611161__/LConn1 -- _CN_92611161_150000_CN_85646787_150000/LConn1
  _CN_92611161_150000_CN_92611154_150000/LConn2 -- T_92611161__/LConn2 -- _CN_92611161_150000_CN_85646787_150000/LConn2
  _CN_92611161_150000_CN_92611154_150000/LConn3 -- T_92611161__/LConn3 -- _CN_92611161_150000_CN_85646787_150000/LConn3 -- bus13/LConn1
  T_92611154__/LConn1 -- _CN_92611161_150000_CN_92611154_150000/RConn1
  T_92611154__/LConn2 -- _CN_92611161_150000_CN_92611154_150000/RConn2
  _CN_92611161_150000_CN_92611154_150000/RConn3 -- T_92611154__/LConn3 -- bus14/LConn1
  _CN_92611161_150000_CN_85646787_150000/RConn1 -- T_85646787__/RConn1 -- _CN_92611147_150000_CN_85646787_150000/LConn1 -- L_85646787/LConn1
  _CN_92611161_150000_CN_85646787_150000/RConn2 -- T_85646787__/RConn2 -- _CN_92611147_150000_CN_85646787_150000/LConn2 -- L_85646787/LConn2
  _CN_92611161_150000_CN_85646787_150000/RConn3 -- T_85646787__/RConn3 -- _CN_92611147_150000_CN_85646787_150000/LConn3 -- L_85646787/LConn3 -- bus15/LConn1
  T_249407518__/LConn1 -- _CN_249407518_150000_CN_196753738_150000/LConn1
  T_249407518__/LConn2 -- _CN_249407518_150000_CN_196753738_150000/LConn2
  _CN_249407518_150000_CN_196753738_150000/LConn3 -- T_249407518__/LConn3 -- bus16/LConn1
  _CN_249407518_150000_CN_196753738_150000/RConn1 -- T_196753738__/LConn1 -- _CN_249407519_150000_CN_196753738_150000/LConn1
  _CN_249407518_150000_CN_196753738_150000/RConn2 -- T_196753738__/LConn2 -- _CN_249407519_150000_CN_196753738_150000/LConn2
  _CN_249407518_150000_CN_196753738_150000/RConn3 -- T_196753738__/LConn3 -- _CN_249407519_150000_CN_196753738_150000/LConn3 -- bus17/LConn1
  _CN_249407519_150000_CN_249407528_150000/LConn1 -- T_249407519__/LConn1 -- _CN_249407519_150000_CN_196753738_150000/RConn1 -- _CN_249407519_150000_CN_140248148_150000/LConn1
  _CN_249407519_150000_CN_249407528_150000/LConn2 -- T_249407519__/LConn2 -- _CN_249407519_150000_CN_196753738_150000/RConn2 -- _CN_249407519_150000_CN_140248148_150000/LConn2
  _CN_249407519_150000_CN_249407528_150000/LConn3 -- T_249407519__/LConn3 -- _CN_249407519_150000_CN_196753738_150000/RConn3 -- _CN_249407519_150000_CN_140248148_150000/LConn3 -- bus18/LConn1
  T_249407528__/LConn1 -- _CN_249407519_150000_CN_249407528_150000/RConn1
  T_249407528__/LConn2 -- _CN_249407519_150000_CN_249407528_150000/RConn2
  _CN_249407519_150000_CN_249407528_150000/RConn3 -- T_249407528__/LConn3 -- bus19/LConn1
  _CN_249407519_150000_CN_140248148_150000/RConn1 -- T_140248148__Κέντρο_Υπερυψηλής_Τάσης_Αράχθου/RConn1 -- _CN_140248148_150000_CN_143520210_150000/LConn1 -- L_140248148/LConn1
  _CN_249407519_150000_CN_140248148_150000/RConn2 -- T_140248148__Κέντρο_Υπερυψηλής_Τάσης_Αράχθου/RConn2 -- _CN_140248148_150000_CN_143520210_150000/LConn2 -- L_140248148/LConn2
  _CN_249407519_150000_CN_140248148_150000/RConn3 -- T_140248148__Κέντρο_Υπερυψηλής_Τάσης_Αράχθου/RConn3 -- _CN_140248148_150000_CN_143520210_150000/LConn3 -- L_140248148/LConn3 -- bus20/LConn1
  T_95989793__/LConn1 -- _CN_95989793_150000_CN_92352843_150000/LConn1
  T_95989793__/LConn2 -- _CN_95989793_150000_CN_92352843_150000/LConn2
  _CN_95989793_150000_CN_92352843_150000/LConn3 -- T_95989793__/LConn3 -- bus21/LConn1
  _CN_95989793_150000_CN_92352843_150000/RConn1 -- T_92352843__/LConn1 -- _CN_51408420_150000_CN_92352843_150000/LConn1 -- _CN_134935126_150000_CN_92352843_150000/LConn1 -- _CN_142174863_150000_CN_92352843_150000/LConn1 -- _CN_92352843_150000_CN_149922043_150000/LConn1
  _CN_95989793_150000_CN_92352843_150000/RConn2 -- T_92352843__/LConn2 -- _CN_51408420_150000_CN_92352843_150000/LConn2 -- _CN_134935126_150000_CN_92352843_150000/LConn2 -- _CN_142174863_150000_CN_92352843_150000/LConn2 -- _CN_92352843_150000_CN_149922043_150000/LConn2
  _CN_95989793_150000_CN_92352843_150000/RConn3 -- T_92352843__/LConn3 -- _CN_51408420_150000_CN_92352843_150000/LConn3 -- _CN_134935126_150000_CN_92352843_150000/LConn3 -- _CN_142174863_150000_CN_92352843_150000/LConn3 -- _CN_92352843_150000_CN_149922043_150000/LConn3 -- bus22/LConn1
  _CN_51408420_150000_CN_134935126_150000/LConn1 -- T_51408420__Κέντρο_Υπερυψηλής_Τάσης_Κουμουνδούρου/RConn1 -- _CN_51408420_150000_CN_93645374_150000/LConn1 -- _CN_51408420_150000_CN_93702884_150000/LConn1 -- _CN_51408420_150000_CN_92352843_150000/RConn1 -- _CN_51408420_150000_CN_134819995_150000/LConn1 -- _CN_51408420_150000_CN_142656551_150000/LConn1 -- Γ_Μ__ΚΥΤ_Διστόμου___ΚΥΤ_Κουμουνδούρου_CN_51408420_150000_CN_85518393_150000/LConn1 -- L_51408420/LConn1
  _CN_51408420_150000_CN_134935126_150000/LConn2 -- T_51408420__Κέντρο_Υπερυψηλής_Τάσης_Κουμουνδούρου/RConn2 -- _CN_51408420_150000_CN_93645374_150000/LConn2 -- _CN_51408420_150000_CN_93702884_150000/LConn2 -- _CN_51408420_150000_CN_92352843_150000/RConn2 -- _CN_51408420_150000_CN_134819995_150000/LConn2 -- _CN_51408420_150000_CN_142656551_150000/LConn2 -- Γ_Μ__ΚΥΤ_Διστόμου___ΚΥΤ_Κουμουνδούρου_CN_51408420_150000_CN_85518393_150000/LConn2 -- L_51408420/LConn2
  _CN_51408420_150000_CN_134935126_150000/LConn3 -- T_51408420__Κέντρο_Υπερυψηλής_Τάσης_Κουμουνδούρου/RConn3 -- _CN_51408420_150000_CN_93645374_150000/LConn3 -- _CN_51408420_150000_CN_93702884_150000/LConn3 -- _CN_51408420_150000_CN_92352843_150000/RConn3 -- _CN_51408420_150000_CN_134819995_150000/LConn3 -- _CN_51408420_150000_CN_142656551_150000/LConn3 -- Γ_Μ__ΚΥΤ_Διστόμου___ΚΥΤ_Κουμουνδούρου_CN_51408420_150000_CN_85518393_150000/LConn3 -- L_51408420/LConn3 -- bus23/LConn1
  _CN_51408420_150000_CN_134935126_150000/RConn1 -- T_134935126__/LConn1 -- _CN_134935126_150000_CN_92352843_150000/RConn1
  _CN_51408420_150000_CN_134935126_150000/RConn2 -- T_134935126__/LConn2 -- _CN_134935126_150000_CN_92352843_150000/RConn2
  _CN_51408420_150000_CN_134935126_150000/RConn3 -- T_134935126__/LConn3 -- _CN_134935126_150000_CN_92352843_150000/RConn3 -- bus24/LConn1
  T_93645374__/LConn1 -- _CN_51408420_150000_CN_93645374_150000/RConn1
  T_93645374__/LConn2 -- _CN_51408420_150000_CN_93645374_150000/RConn2
  _CN_51408420_150000_CN_93645374_150000/RConn3 -- T_93645374__/LConn3 -- bus25/LConn1
  T_93702884__/LConn1 -- _CN_51408420_150000_CN_93702884_150000/RConn1
  T_93702884__/LConn2 -- _CN_51408420_150000_CN_93702884_150000/RConn2
  _CN_51408420_150000_CN_93702884_150000/RConn3 -- T_93702884__/LConn3 -- bus26/LConn1
  T_134819995__/LConn1 -- _CN_51408420_150000_CN_134819995_150000/RConn1
  T_134819995__/LConn2 -- _CN_51408420_150000_CN_134819995_150000/RConn2
  _CN_51408420_150000_CN_134819995_150000/RConn3 -- T_134819995__/LConn3 -- bus27/LConn1
  T_142656551__/LConn1 -- _CN_51408420_150000_CN_142656551_150000/RConn1
  T_142656551__/LConn2 -- _CN_51408420_150000_CN_142656551_150000/RConn2
  _CN_51408420_150000_CN_142656551_150000/RConn3 -- T_142656551__/LConn3 -- bus28/LConn1
  Γ_Μ__ΚΥΤ_Διστόμου___ΚΥΤ_Κουμουνδούρου_CN_51408420_150000_CN_85518393_150000/RConn1 -- T_85518393__Κέντρο_Υπερυψηλής_Τάσης_Διστόμου/RConn1 -- L_85518393/LConn1
  Γ_Μ__ΚΥΤ_Διστόμου___ΚΥΤ_Κουμουνδούρου_CN_51408420_150000_CN_85518393_150000/RConn2 -- T_85518393__Κέντρο_Υπερυψηλής_Τάσης_Διστόμου/RConn2 -- L_85518393/LConn2
  Γ_Μ__ΚΥΤ_Διστόμου___ΚΥΤ_Κουμουνδούρου_CN_51408420_150000_CN_85518393_150000/RConn3 -- T_85518393__Κέντρο_Υπερυψηλής_Τάσης_Διστόμου/RConn3 -- L_85518393/LConn3 -- bus29/LConn1
  _CN_140637735_150000_CN_140724364_150000/LConn1 -- T_140637735__/LConn1 -- _CN_140637735_150000_CN_140890157_150000/LConn1
  _CN_140637735_150000_CN_140724364_150000/LConn2 -- T_140637735__/LConn2 -- _CN_140637735_150000_CN_140890157_150000/LConn2
  _CN_140637735_150000_CN_140724364_150000/LConn3 -- T_140637735__/LConn3 -- _CN_140637735_150000_CN_140890157_150000/LConn3 -- bus30/LConn1
  _CN_140637735_150000_CN_140724364_150000/RConn1 -- T_140724364__/LConn1 -- _CN_140724364_150000_CN_141113249_150000/LConn1 -- _CN_140724364_150000_CN_118901197_150000/LConn1
  _CN_140637735_150000_CN_140724364_150000/RConn2 -- T_140724364__/LConn2 -- _CN_140724364_150000_CN_141113249_150000/LConn2 -- _CN_140724364_150000_CN_118901197_150000/LConn2
  _CN_140637735_150000_CN_140724364_150000/RConn3 -- T_140724364__/LConn3 -- _CN_140724364_150000_CN_141113249_150000/LConn3 -- _CN_140724364_150000_CN_118901197_150000/LConn3 -- bus31/LConn1
  T_140890157__/LConn1 -- _CN_140637735_150000_CN_140890157_150000/RConn1
  T_140890157__/LConn2 -- _CN_140637735_150000_CN_140890157_150000/RConn2
  _CN_140637735_150000_CN_140890157_150000/RConn3 -- T_140890157__/LConn3 -- bus32/LConn1
  T_135463990__/LConn1 -- _CN_135463990_150000_CN_93061390_150000/LConn1
  T_135463990__/LConn2 -- _CN_135463990_150000_CN_93061390_150000/LConn2
  _CN_135463990_150000_CN_93061390_150000/LConn3 -- T_135463990__/LConn3 -- bus33/LConn1
  _CN_135463990_150000_CN_93061390_150000/RConn1 -- T_93061390__/LConn1 -- _CN_85526073_150000_CN_93061390_150000/LConn1 -- _CN_93085804_150000_CN_93061390_150000/LConn1 -- _CN_93061385_150000_CN_93061390_150000/LConn1 -- _CN_93061390_150000_CN_115027244_150000/LConn1
  _CN_135463990_150000_CN_93061390_150000/RConn2 -- T_93061390__/LConn2 -- _CN_85526073_150000_CN_93061390_150000/LConn2 -- _CN_93085804_150000_CN_93061390_150000/LConn2 -- _CN_93061385_150000_CN_93061390_150000/LConn2 -- _CN_93061390_150000_CN_115027244_150000/LConn2
  _CN_135463990_150000_CN_93061390_150000/RConn3 -- T_93061390__/LConn3 -- _CN_85526073_150000_CN_93061390_150000/LConn3 -- _CN_93085804_150000_CN_93061390_150000/LConn3 -- _CN_93061385_150000_CN_93061390_150000/LConn3 -- _CN_93061390_150000_CN_115027244_150000/LConn3 -- bus34/LConn1
  _CN_85526073_150000_CN_135177715_150000/LConn1 -- T_85526073__/RConn1 -- _CN_85526073_150000_CN_93061390_150000/RConn1 -- L_85526073/LConn1
  _CN_85526073_150000_CN_135177715_150000/LConn2 -- T_85526073__/RConn2 -- _CN_85526073_150000_CN_93061390_150000/RConn2 -- L_85526073/LConn2
  _CN_85526073_150000_CN_135177715_150000/LConn3 -- T_85526073__/RConn3 -- _CN_85526073_150000_CN_93061390_150000/RConn3 -- L_85526073/LConn3 -- bus35/LConn1
  _CN_85526073_150000_CN_135177715_150000/RConn1 -- T_135177715__ΥΠΟΣΤΑΘΜΟΣ__Δ_Ε_Η_/LConn1 -- _CN_143622720_150000_CN_135177715_150000/LConn1 -- _CN_86577898_150000_CN_135177715_150000/LConn1 -- _CN_219975140_150000_CN_135177715_150000/LConn1 -- _CN_135177715_150000_CN_93172457_150000/LConn1 -- _CN_248889404_150000_CN_135177715_150000/LConn1
  _CN_85526073_150000_CN_135177715_150000/RConn2 -- T_135177715__ΥΠΟΣΤΑΘΜΟΣ__Δ_Ε_Η_/LConn2 -- _CN_143622720_150000_CN_135177715_150000/LConn2 -- _CN_86577898_150000_CN_135177715_150000/LConn2 -- _CN_219975140_150000_CN_135177715_150000/LConn2 -- _CN_135177715_150000_CN_93172457_150000/LConn2 -- _CN_248889404_150000_CN_135177715_150000/LConn2
  _CN_85526073_150000_CN_135177715_150000/RConn3 -- T_135177715__ΥΠΟΣΤΑΘΜΟΣ__Δ_Ε_Η_/LConn3 -- _CN_143622720_150000_CN_135177715_150000/LConn3 -- _CN_86577898_150000_CN_135177715_150000/LConn3 -- _CN_219975140_150000_CN_135177715_150000/LConn3 -- _CN_135177715_150000_CN_93172457_150000/LConn3 -- bus36/LConn1 -- _CN_248889404_150000_CN_135177715_150000/LConn3
  _CN_128088635_150000_CN_93073613_150000/LConn1 -- T_128088635__/LConn1 -- _CN_128088635_150000_CN_136549173_150000/LConn1
  _CN_128088635_150000_CN_93073613_150000/LConn2 -- T_128088635__/LConn2 -- _CN_128088635_150000_CN_136549173_150000/LConn2
  _CN_128088635_150000_CN_93073613_150000/LConn3 -- T_128088635__/LConn3 -- _CN_128088635_150000_CN_136549173_150000/LConn3 -- bus37/LConn1
  T_93073613__/LConn1 -- _CN_128088635_150000_CN_93073613_150000/RConn1
  T_93073613__/LConn2 -- _CN_128088635_150000_CN_93073613_150000/RConn2
  _CN_128088635_150000_CN_93073613_150000/RConn3 -- T_93073613__/LConn3 -- bus38/LConn1
  T_136549173__/LConn1 -- _CN_128088635_150000_CN_136549173_150000/RConn1
  T_136549173__/LConn2 -- _CN_128088635_150000_CN_136549173_150000/RConn2
  _CN_128088635_150000_CN_136549173_150000/RConn3 -- T_136549173__/LConn3 -- bus39/LConn1
  _CN_248889404_150000_CN_136549175_150000/LConn1 -- T_248889404__/LConn1 -- _CN_248889404_150000_CN_135177715_150000/RConn1 -- _CN_248889404_150000_CN_136543640_150000/LConn1
  _CN_248889404_150000_CN_136549175_150000/LConn2 -- T_248889404__/LConn2 -- _CN_248889404_150000_CN_135177715_150000/RConn2 -- _CN_248889404_150000_CN_136543640_150000/LConn2
  _CN_248889404_150000_CN_136549175_150000/LConn3 -- T_248889404__/LConn3 -- _CN_248889404_150000_CN_135177715_150000/RConn3 -- bus40/LConn1 -- _CN_248889404_150000_CN_136543640_150000/LConn3
  _CN_248889404_150000_CN_136549175_150000/RConn1 -- T_136549175__/LConn1 -- _CN_136549175_150000_CN_136549181_150000/LConn1
  _CN_248889404_150000_CN_136549175_150000/RConn2 -- T_136549175__/LConn2 -- _CN_136549175_150000_CN_136549181_150000/LConn2
  _CN_248889404_150000_CN_136549175_150000/RConn3 -- T_136549175__/LConn3 -- _CN_136549175_150000_CN_136549181_150000/LConn3 -- bus41/LConn1
  _CN_248889404_150000_CN_136543640_150000/RConn1 -- T_136543640__/LConn1 -- _CN_86577898_150000_CN_136543640_150000/LConn1 -- _CN_136543640_150000_CN_136369149_150000/LConn1
  _CN_248889404_150000_CN_136543640_150000/RConn2 -- T_136543640__/LConn2 -- _CN_86577898_150000_CN_136543640_150000/LConn2 -- _CN_136543640_150000_CN_136369149_150000/LConn2
  _CN_248889404_150000_CN_136543640_150000/RConn3 -- T_136543640__/LConn3 -- _CN_86577898_150000_CN_136543640_150000/LConn3 -- _CN_136543640_150000_CN_136369149_150000/LConn3 -- bus42/LConn1
  T_134630651__/LConn1 -- _CN_85612093_150000_CN_134630651_150000/RConn1
  T_134630651__/LConn2 -- _CN_85612093_150000_CN_134630651_150000/RConn2
  _CN_85612093_150000_CN_134630651_150000/RConn3 -- T_134630651__/LConn3 -- bus43/LConn1
  T_93583004__/LConn1 -- _CN_85612093_150000_CN_93583004_150000/RConn1
  T_93583004__/LConn2 -- _CN_85612093_150000_CN_93583004_150000/RConn2
  _CN_85612093_150000_CN_93583004_150000/RConn3 -- T_93583004__/LConn3 -- bus44/LConn1
  T_86466243__Υ_Σ_Ανατολής/LConn1 -- _CN_85612093_150000_CN_86466243_150000/RConn1
  T_86466243__Υ_Σ_Ανατολής/LConn2 -- _CN_85612093_150000_CN_86466243_150000/RConn2
  _CN_85612093_150000_CN_86466243_150000/RConn3 -- T_86466243__Υ_Σ_Ανατολής/LConn3 -- bus45/LConn1
  _CN_143622720_150000_CN_135177715_150000/RConn1 -- T_143622720__/LConn1 -- _CN_143622720_150000_CN_105184051_150000/LConn1
  _CN_143622720_150000_CN_135177715_150000/RConn2 -- T_143622720__/LConn2 -- _CN_143622720_150000_CN_105184051_150000/LConn2
  _CN_143622720_150000_CN_135177715_150000/RConn3 -- T_143622720__/LConn3 -- _CN_143622720_150000_CN_105184051_150000/LConn3 -- bus46/LConn1
  _CN_143622720_150000_CN_105184051_150000/RConn1 -- T_105184051_400000;150000_Κέντρο_Υπερυψηλής_Τάσης_Αχελώου/RConn1 -- _CN_249108719_150000_CN_105184051_150000/LConn1 -- _CN_105184051_150000_CN_143520210_150000/LConn1 -- L_105184051/LConn1
  _CN_143622720_150000_CN_105184051_150000/RConn2 -- T_105184051_400000;150000_Κέντρο_Υπερυψηλής_Τάσης_Αχελώου/RConn2 -- _CN_249108719_150000_CN_105184051_150000/LConn2 -- _CN_105184051_150000_CN_143520210_150000/LConn2 -- L_105184051/LConn2
  _CN_143622720_150000_CN_105184051_150000/RConn3 -- T_105184051_400000;150000_Κέντρο_Υπερυψηλής_Τάσης_Αχελώου/RConn3 -- _CN_249108719_150000_CN_105184051_150000/LConn3 -- _CN_105184051_150000_CN_143520210_150000/LConn3 -- L_105184051/LConn3 -- bus47/LConn1
  _CN_120740424_150000_CN_128799211_150000/LConn1 -- T_120740424__/LConn1 -- _CN_120740424_150000_CN_141764450_150000/LConn1
  _CN_120740424_150000_CN_128799211_150000/LConn2 -- T_120740424__/LConn2 -- _CN_120740424_150000_CN_141764450_150000/LConn2
  _CN_120740424_150000_CN_128799211_150000/LConn3 -- T_120740424__/LConn3 -- _CN_120740424_150000_CN_141764450_150000/LConn3 -- bus48/LConn1
  _CN_120740424_150000_CN_128799211_150000/RConn1 -- T_128799211__/LConn1 -- _CN_96759614_150000_CN_128799211_150000/LConn1
  _CN_120740424_150000_CN_128799211_150000/RConn2 -- T_128799211__/LConn2 -- _CN_96759614_150000_CN_128799211_150000/LConn2
  _CN_120740424_150000_CN_128799211_150000/RConn3 -- T_128799211__/LConn3 -- _CN_96759614_150000_CN_128799211_150000/LConn3 -- bus49/LConn1
  T_141764450__/LConn1 -- _CN_120740424_150000_CN_141764450_150000/RConn1
  T_141764450__/LConn2 -- _CN_120740424_150000_CN_141764450_150000/RConn2
  _CN_120740424_150000_CN_141764450_150000/RConn3 -- T_141764450__/LConn3 -- bus50/LConn1
  T_92611147__/LConn1 -- _CN_92611147_150000_CN_85646787_150000/RConn1
  T_92611147__/LConn2 -- _CN_92611147_150000_CN_85646787_150000/RConn2
  _CN_92611147_150000_CN_85646787_150000/RConn3 -- T_92611147__/LConn3 -- bus51/LConn1
  T_249414224__/LConn1 -- _CN_249414224_150000_CN_120913153_150000/LConn1
  T_249414224__/LConn2 -- _CN_249414224_150000_CN_120913153_150000/LConn2
  _CN_249414224_150000_CN_120913153_150000/LConn3 -- T_249414224__/LConn3 -- bus52/LConn1
  _CN_249414224_150000_CN_120913153_150000/RConn1 -- T_120913153__/LConn1 -- _CN_249407521_150000_CN_120913153_150000/LConn1
  _CN_249414224_150000_CN_120913153_150000/RConn2 -- T_120913153__/LConn2 -- _CN_249407521_150000_CN_120913153_150000/LConn2
  _CN_249414224_150000_CN_120913153_150000/RConn3 -- T_120913153__/LConn3 -- _CN_249407521_150000_CN_120913153_150000/LConn3 -- bus53/LConn1
  _CN_142066771_150000_CN_142066784_150000/LConn1 -- T_142066771__/LConn1 -- _CN_142066771_150000_CN_178234508_150000/LConn1
  _CN_142066771_150000_CN_142066784_150000/LConn2 -- T_142066771__/LConn2 -- _CN_142066771_150000_CN_178234508_150000/LConn2
  _CN_142066771_150000_CN_142066784_150000/LConn3 -- T_142066771__/LConn3 -- _CN_142066771_150000_CN_178234508_150000/LConn3 -- bus54/LConn1
  T_142066784__/LConn1 -- _CN_142066771_150000_CN_142066784_150000/RConn1
  T_142066784__/LConn2 -- _CN_142066771_150000_CN_142066784_150000/RConn2
  _CN_142066771_150000_CN_142066784_150000/RConn3 -- T_142066784__/LConn3 -- bus55/LConn1
  T_178234508__/LConn1 -- _CN_142066771_150000_CN_178234508_150000/RConn1
  T_178234508__/LConn2 -- _CN_142066771_150000_CN_178234508_150000/RConn2
  _CN_142066771_150000_CN_178234508_150000/RConn3 -- T_178234508__/LConn3 -- bus56/LConn1
  _CN_140248148_150000_CN_143520210_150000/RConn1 -- T_143520210__/LConn1 -- _CN_105184051_150000_CN_143520210_150000/RConn1 -- _CN_135266022_150000_CN_143520210_150000/LConn1
  _CN_140248148_150000_CN_143520210_150000/RConn2 -- T_143520210__/LConn2 -- _CN_105184051_150000_CN_143520210_150000/RConn2 -- _CN_135266022_150000_CN_143520210_150000/LConn2
  _CN_140248148_150000_CN_143520210_150000/RConn3 -- T_143520210__/LConn3 -- _CN_105184051_150000_CN_143520210_150000/RConn3 -- bus57/LConn1 -- _CN_135266022_150000_CN_143520210_150000/LConn3
  T_93085785__/LConn1 -- _CN_93085785_150000_CN_93085804_150000/LConn1
  T_93085785__/LConn2 -- _CN_93085785_150000_CN_93085804_150000/LConn2
  _CN_93085785_150000_CN_93085804_150000/LConn3 -- T_93085785__/LConn3 -- bus58/LConn1
  _CN_93085785_150000_CN_93085804_150000/RConn1 -- T_93085804__/LConn1 -- _CN_93085804_150000_CN_93061390_150000/RConn1
  _CN_93085785_150000_CN_93085804_150000/RConn2 -- T_93085804__/LConn2 -- _CN_93085804_150000_CN_93061390_150000/RConn2
  _CN_93085785_150000_CN_93085804_150000/RConn3 -- T_93085804__/LConn3 -- _CN_93085804_150000_CN_93061390_150000/RConn3 -- bus59/LConn1
  _CN_279628389_150000_CN_148899598_150000/LConn1 -- T_279628389__/LConn1 -- _CN_279628389_150000_CN_149026603_150000/LConn1 -- _CN_279628389_150000_CN_55099563_150000/RConn1
  _CN_279628389_150000_CN_148899598_150000/LConn2 -- T_279628389__/LConn2 -- _CN_279628389_150000_CN_149026603_150000/LConn2 -- _CN_279628389_150000_CN_55099563_150000/RConn2
  _CN_279628389_150000_CN_148899598_150000/LConn3 -- T_279628389__/LConn3 -- _CN_279628389_150000_CN_149026603_150000/LConn3 -- bus60/LConn1 -- _CN_279628389_150000_CN_55099563_150000/RConn3
  _CN_279628389_150000_CN_148899598_150000/RConn1 -- T_148899598__/LConn1 -- _CN_149069221_150000_CN_148899598_150000/LConn1 -- _CN_148899591_150000_CN_148899598_150000/LConn1
  _CN_279628389_150000_CN_148899598_150000/RConn2 -- T_148899598__/LConn2 -- _CN_149069221_150000_CN_148899598_150000/LConn2 -- _CN_148899591_150000_CN_148899598_150000/LConn2
  _CN_279628389_150000_CN_148899598_150000/RConn3 -- T_148899598__/LConn3 -- _CN_149069221_150000_CN_148899598_150000/LConn3 -- bus61/LConn1 -- _CN_148899591_150000_CN_148899598_150000/LConn3
  _CN_279628389_150000_CN_149026603_150000/RConn1 -- T_149026603__/LConn1 -- _CN_149026599_150000_CN_149026603_150000/LConn1
  _CN_279628389_150000_CN_149026603_150000/RConn2 -- T_149026603__/LConn2 -- _CN_149026599_150000_CN_149026603_150000/LConn2
  _CN_279628389_150000_CN_149026603_150000/RConn3 -- T_149026603__/LConn3 -- _CN_149026599_150000_CN_149026603_150000/LConn3 -- bus62/LConn1
  T_141514344__/LConn1 -- _CN_141514344_150000_CN_55099563_150000/RConn1
  T_141514344__/LConn2 -- _CN_141514344_150000_CN_55099563_150000/RConn2
  _CN_141514344_150000_CN_55099563_150000/RConn3 -- T_141514344__/LConn3 -- bus63/LConn1
  T_148881241__/LConn1 -- _CN_148881241_150000_CN_129452806_150000/LConn1
  T_148881241__/LConn2 -- _CN_148881241_150000_CN_129452806_150000/LConn2
  _CN_148881241_150000_CN_129452806_150000/LConn3 -- T_148881241__/LConn3 -- bus64/LConn1
  _CN_148881241_150000_CN_129452806_150000/RConn1 -- T_129452806__/LConn1 -- _CN_129452806_150000_CN_129452815_150000/LConn1 -- _CN_86577898_150000_CN_129452806_150000/LConn1
  _CN_148881241_150000_CN_129452806_150000/RConn2 -- T_129452806__/LConn2 -- _CN_129452806_150000_CN_129452815_150000/LConn2 -- _CN_86577898_150000_CN_129452806_150000/LConn2
  _CN_148881241_150000_CN_129452806_150000/RConn3 -- T_129452806__/LConn3 -- _CN_129452806_150000_CN_129452815_150000/LConn3 -- bus65/LConn1 -- _CN_86577898_150000_CN_129452806_150000/LConn3
  T_252802673__/LConn1 -- _CN_252802673_150000_CN_15642023_150000/RConn1
  T_252802673__/LConn2 -- _CN_252802673_150000_CN_15642023_150000/RConn2
  _CN_252802673_150000_CN_15642023_150000/RConn3 -- T_252802673__/LConn3 -- bus66/LConn1
  T_142180032__/LConn1 -- _CN_142180032_150000_CN_142174863_150000/LConn1
  T_142180032__/LConn2 -- _CN_142180032_150000_CN_142174863_150000/LConn2
  _CN_142180032_150000_CN_142174863_150000/LConn3 -- T_142180032__/LConn3 -- bus67/LConn1
  _CN_142180032_150000_CN_142174863_150000/RConn1 -- T_142174863__/LConn1 -- _CN_142174863_150000_CN_92352843_150000/RConn1 -- _CN_142174863_150000_CN_253912195_150000/LConn1
  _CN_142180032_150000_CN_142174863_150000/RConn2 -- T_142174863__/LConn2 -- _CN_142174863_150000_CN_92352843_150000/RConn2 -- _CN_142174863_150000_CN_253912195_150000/LConn2
  _CN_142180032_150000_CN_142174863_150000/RConn3 -- T_142174863__/LConn3 -- _CN_142174863_150000_CN_92352843_150000/RConn3 -- _CN_142174863_150000_CN_253912195_150000/LConn3 -- bus68/LConn1
  T_128870336__/LConn1 -- _CN_128870336_150000_CN_148320053_150000/LConn1
  T_128870336__/LConn2 -- _CN_128870336_150000_CN_148320053_150000/LConn2
  _CN_128870336_150000_CN_148320053_150000/LConn3 -- T_128870336__/LConn3 -- bus69/LConn1
  T_148320053__/LConn1 -- _CN_128870336_150000_CN_148320053_150000/RConn1
  T_148320053__/LConn2 -- _CN_128870336_150000_CN_148320053_150000/RConn2
  _CN_128870336_150000_CN_148320053_150000/RConn3 -- T_148320053__/LConn3 -- bus70/LConn1
  _CN_141685890_150000_CN_93885376_150000/LConn1 -- T_141685890__/LConn1 -- _CN_141685890_150000_CN_141685891_150000/LConn1
  _CN_141685890_150000_CN_93885376_150000/LConn2 -- T_141685890__/LConn2 -- _CN_141685890_150000_CN_141685891_150000/LConn2
  _CN_141685890_150000_CN_93885376_150000/LConn3 -- T_141685890__/LConn3 -- _CN_141685890_150000_CN_141685891_150000/LConn3 -- bus71/LConn1
  T_93885376__/LConn1 -- _CN_141685890_150000_CN_93885376_150000/RConn1
  T_93885376__/LConn2 -- _CN_141685890_150000_CN_93885376_150000/RConn2
  _CN_141685890_150000_CN_93885376_150000/RConn3 -- T_93885376__/LConn3 -- bus72/LConn1
  T_141685891__/LConn1 -- _CN_141685890_150000_CN_141685891_150000/RConn1
  T_141685891__/LConn2 -- _CN_141685890_150000_CN_141685891_150000/RConn2
  _CN_141685890_150000_CN_141685891_150000/RConn3 -- T_141685891__/LConn3 -- bus73/LConn1
  T_141113249__/LConn1 -- _CN_140724364_150000_CN_141113249_150000/RConn1
  T_141113249__/LConn2 -- _CN_140724364_150000_CN_141113249_150000/RConn2
  _CN_140724364_150000_CN_141113249_150000/RConn3 -- T_141113249__/LConn3 -- bus74/LConn1
  _CN_140724364_150000_CN_118901197_150000/RConn1 -- G_118901197_/RConn1 -- _CN_141029834_150000_CN_118901197_150000/LConn1
  _CN_140724364_150000_CN_118901197_150000/RConn2 -- G_118901197_/RConn2 -- _CN_141029834_150000_CN_118901197_150000/LConn2
  _CN_140724364_150000_CN_118901197_150000/RConn3 -- G_118901197_/RConn3 -- _CN_141029834_150000_CN_118901197_150000/LConn3 -- bus75/LConn1
  T_141533837__/LConn1 -- _CN_141533837_150000_CN_141533838_150000/LConn1
  T_141533837__/LConn2 -- _CN_141533837_150000_CN_141533838_150000/LConn2
  _CN_141533837_150000_CN_141533838_150000/LConn3 -- T_141533837__/LConn3 -- bus76/LConn1
  T_141533838__/LConn1 -- _CN_141533837_150000_CN_141533838_150000/RConn1
  T_141533838__/LConn2 -- _CN_141533837_150000_CN_141533838_150000/RConn2
  _CN_141533837_150000_CN_141533838_150000/RConn3 -- T_141533838__/LConn3 -- bus77/LConn1
  _CN_142174863_150000_CN_253912195_150000/RConn1 -- T_253912195__/LConn1 -- _CN_254057189_150000_CN_253912195_150000/LConn1
  _CN_142174863_150000_CN_253912195_150000/RConn2 -- T_253912195__/LConn2 -- _CN_254057189_150000_CN_253912195_150000/LConn2
  _CN_142174863_150000_CN_253912195_150000/RConn3 -- T_253912195__/LConn3 -- _CN_254057189_150000_CN_253912195_150000/LConn3 -- bus78/LConn1
  T_149468818__/LConn1 -- _CN_149468818_150000_CN_149481032_150000/LConn1
  T_149468818__/LConn2 -- _CN_149468818_150000_CN_149481032_150000/LConn2
  _CN_149468818_150000_CN_149481032_150000/LConn3 -- T_149468818__/LConn3 -- bus79/LConn1
  _CN_149468818_150000_CN_149481032_150000/RConn1 -- T_149481032__/LConn1 -- _CN_149481032_150000_CN_93172457_150000/LConn1
  _CN_149468818_150000_CN_149481032_150000/RConn2 -- T_149481032__/LConn2 -- _CN_149481032_150000_CN_93172457_150000/LConn2
  _CN_149468818_150000_CN_149481032_150000/RConn3 -- T_149481032__/LConn3 -- _CN_149481032_150000_CN_93172457_150000/LConn3 -- bus80/LConn1
  T_254347424__/LConn1 -- _CN_254347424_150000_CN_136370140_150000/LConn1
  T_254347424__/LConn2 -- _CN_254347424_150000_CN_136370140_150000/LConn2
  _CN_254347424_150000_CN_136370140_150000/LConn3 -- T_254347424__/LConn3 -- bus81/LConn1
  _CN_254347424_150000_CN_136370140_150000/RConn1 -- T_136370140__/LConn1 -- _CN_86577898_150000_CN_136370140_150000/LConn1
  _CN_254347424_150000_CN_136370140_150000/RConn2 -- T_136370140__/LConn2 -- _CN_86577898_150000_CN_136370140_150000/LConn2
  _CN_254347424_150000_CN_136370140_150000/RConn3 -- T_136370140__/LConn3 -- _CN_86577898_150000_CN_136370140_150000/LConn3 -- bus82/LConn1
  T_159413454__/LConn1 -- _CN_55099563_150000_CN_159413454_150000/RConn1
  T_159413454__/LConn2 -- _CN_55099563_150000_CN_159413454_150000/RConn2
  _CN_55099563_150000_CN_159413454_150000/RConn3 -- T_159413454__/LConn3 -- bus83/LConn1
  T_92508649__/LConn1 -- _CN_55099563_150000_CN_92508649_150000/RConn1
  T_92508649__/LConn2 -- _CN_55099563_150000_CN_92508649_150000/RConn2
  _CN_55099563_150000_CN_92508649_150000/RConn3 -- T_92508649__/LConn3 -- bus84/LConn1
  T_92508651__Υποσταθμός_Δόξας/LConn1 -- _CN_55099563_150000_CN_92508651_150000/RConn1
  T_92508651__Υποσταθμός_Δόξας/LConn2 -- _CN_55099563_150000_CN_92508651_150000/RConn2
  _CN_55099563_150000_CN_92508651_150000/RConn3 -- T_92508651__Υποσταθμός_Δόξας/LConn3 -- bus85/LConn1
  T_141029834__/LConn1 -- _CN_141029834_150000_CN_118901197_150000/RConn1
  T_141029834__/LConn2 -- _CN_141029834_150000_CN_118901197_150000/RConn2
  _CN_141029834_150000_CN_118901197_150000/RConn3 -- T_141029834__/LConn3 -- bus86/LConn1
  T_249407521__Υδροηλεκτρικό_Εργοστάσιο_Λάδωνα/LConn1 -- _CN_249407521_150000_CN_120913153_150000/RConn1
  T_249407521__Υδροηλεκτρικό_Εργοστάσιο_Λάδωνα/LConn2 -- _CN_249407521_150000_CN_120913153_150000/RConn2
  _CN_249407521_150000_CN_120913153_150000/RConn3 -- T_249407521__Υδροηλεκτρικό_Εργοστάσιο_Λάδωνα/LConn3 -- bus87/LConn1
  T_159413450__/LConn1 -- _CN_159413450_150000_CN_159413451_150000/LConn1
  T_159413450__/LConn2 -- _CN_159413450_150000_CN_159413451_150000/LConn2
  _CN_159413450_150000_CN_159413451_150000/LConn3 -- T_159413450__/LConn3 -- bus88/LConn1
  T_159413451__/LConn1 -- _CN_159413450_150000_CN_159413451_150000/RConn1
  T_159413451__/LConn2 -- _CN_159413450_150000_CN_159413451_150000/RConn2
  _CN_159413450_150000_CN_159413451_150000/RConn3 -- T_159413451__/LConn3 -- bus89/LConn1
  T_254057189__/LConn1 -- _CN_254057189_150000_CN_253912195_150000/RConn1
  T_254057189__/LConn2 -- _CN_254057189_150000_CN_253912195_150000/RConn2
  _CN_254057189_150000_CN_253912195_150000/RConn3 -- T_254057189__/LConn3 -- bus90/LConn1
  _CN_135266022_150000_CN_143520210_150000/RConn1 -- T_135266022__/LConn1 -- _CN_135266022_150000_CN_96040682_150000/LConn1
  _CN_135266022_150000_CN_143520210_150000/RConn2 -- T_135266022__/LConn2 -- _CN_135266022_150000_CN_96040682_150000/LConn2
  _CN_135266022_150000_CN_143520210_150000/RConn3 -- T_135266022__/LConn3 -- _CN_135266022_150000_CN_96040682_150000/LConn3 -- bus91/LConn1
  _CN_135266022_150000_CN_96040682_150000/RConn1 -- T_96040682__/LConn1 -- _CN_96040696_150000_CN_96040682_150000/LConn1
  _CN_135266022_150000_CN_96040682_150000/RConn2 -- T_96040682__/LConn2 -- _CN_96040696_150000_CN_96040682_150000/LConn2
  _CN_135266022_150000_CN_96040682_150000/RConn3 -- T_96040682__/LConn3 -- _CN_96040696_150000_CN_96040682_150000/LConn3 -- bus92/LConn1
  _CN_86577898_150000_CN_129452806_150000/RConn1 -- T_86577898__/RConn1 -- _CN_86577898_150000_CN_136450393_150000/LConn1 -- _CN_86577898_150000_CN_136370140_150000/RConn1 -- L_86577898/LConn1 -- _CN_86577898_150000_CN_135177715_150000/RConn1 -- _CN_86577898_150000_CN_129452812_150000/LConn1 -- _CN_86577898_150000_CN_136543640_150000/RConn1
  _CN_86577898_150000_CN_129452806_150000/RConn2 -- T_86577898__/RConn2 -- _CN_86577898_150000_CN_136450393_150000/LConn2 -- _CN_86577898_150000_CN_136370140_150000/RConn2 -- L_86577898/LConn2 -- _CN_86577898_150000_CN_135177715_150000/RConn2 -- _CN_86577898_150000_CN_129452812_150000/LConn2 -- _CN_86577898_150000_CN_136543640_150000/RConn2
  _CN_86577898_150000_CN_129452806_150000/RConn3 -- T_86577898__/RConn3 -- _CN_86577898_150000_CN_136450393_150000/LConn3 -- _CN_86577898_150000_CN_136370140_150000/RConn3 -- L_86577898/LConn3 -- bus93/LConn1 -- _CN_86577898_150000_CN_135177715_150000/RConn3 -- _CN_86577898_150000_CN_129452812_150000/LConn3 -- _CN_86577898_150000_CN_136543640_150000/RConn3
  _CN_86577898_150000_CN_129452812_150000/RConn1 -- T_129452812__/LConn1 -- _CN_129452812_150000_CN_129452815_150000/LConn1
  _CN_86577898_150000_CN_129452812_150000/RConn2 -- T_129452812__/LConn2 -- _CN_129452812_150000_CN_129452815_150000/LConn2
  _CN_86577898_150000_CN_129452812_150000/RConn3 -- T_129452812__/LConn3 -- _CN_129452812_150000_CN_129452815_150000/LConn3 -- bus94/LConn1
  T_136450393__/LConn1 -- _CN_86577898_150000_CN_136450393_150000/RConn1
  T_136450393__/LConn2 -- _CN_86577898_150000_CN_136450393_150000/RConn2
  _CN_86577898_150000_CN_136450393_150000/RConn3 -- T_136450393__/LConn3 -- bus95/LConn1
  T_249108719__/LConn1 -- _CN_249108719_150000_CN_105184051_150000/RConn1
  T_249108719__/LConn2 -- _CN_249108719_150000_CN_105184051_150000/RConn2
  _CN_249108719_150000_CN_105184051_150000/RConn3 -- T_249108719__/LConn3 -- bus96/LConn1
  _CN_96040696_150000_CN_96040682_150000/RConn1 -- T_96040696__/LConn1 -- _CN_96040696_150000_CN_96314286_150000/LConn1 -- _CN_96040696_150000_CN_96314284_150000/LConn1 -- _CN_96040696_150000_CN_96314289_150000/RConn1
  _CN_96040696_150000_CN_96040682_150000/RConn2 -- T_96040696__/LConn2 -- _CN_96040696_150000_CN_96314286_150000/LConn2 -- _CN_96040696_150000_CN_96314284_150000/LConn2 -- _CN_96040696_150000_CN_96314289_150000/RConn2
  _CN_96040696_150000_CN_96040682_150000/RConn3 -- T_96040696__/LConn3 -- _CN_96040696_150000_CN_96314286_150000/LConn3 -- _CN_96040696_150000_CN_96314284_150000/LConn3 -- _CN_96040696_150000_CN_96314289_150000/RConn3 -- bus97/LConn1
  _CN_96040696_150000_CN_96314286_150000/RConn1 -- T_96314286__/LConn1 -- _CN_96314286_150000_CN_96314289_150000/RConn1
  _CN_96040696_150000_CN_96314286_150000/RConn2 -- T_96314286__/LConn2 -- _CN_96314286_150000_CN_96314289_150000/RConn2
  _CN_96040696_150000_CN_96314286_150000/RConn3 -- T_96314286__/LConn3 -- _CN_96314286_150000_CN_96314289_150000/RConn3 -- bus98/LConn1
  T_96314284__/LConn1 -- _CN_96040696_150000_CN_96314284_150000/RConn1
  T_96314284__/LConn2 -- _CN_96040696_150000_CN_96314284_150000/RConn2
  _CN_96040696_150000_CN_96314284_150000/RConn3 -- T_96314284__/LConn3 -- bus99/LConn1
  T_149922042__/LConn1 -- _CN_149922042_150000_CN_149922043_150000/LConn1
  T_149922042__/LConn2 -- _CN_149922042_150000_CN_149922043_150000/LConn2
  _CN_149922042_150000_CN_149922043_150000/LConn3 -- T_149922042__/LConn3 -- bus100/LConn1
  _CN_149922042_150000_CN_149922043_150000/RConn1 -- T_149922043__/LConn1 -- _CN_92352843_150000_CN_149922043_150000/RConn1
  _CN_149922042_150000_CN_149922043_150000/RConn2 -- T_149922043__/LConn2 -- _CN_92352843_150000_CN_149922043_150000/RConn2
  _CN_149922042_150000_CN_149922043_150000/RConn3 -- T_149922043__/LConn3 -- _CN_92352843_150000_CN_149922043_150000/RConn3 -- bus101/LConn1
  _CN_148899588_150000_CN_149069221_150000/LConn1 -- T_148899588__/LConn1 -- _CN_148899588_150000_CN_93173562_150000/LConn1
  _CN_148899588_150000_CN_149069221_150000/LConn2 -- T_148899588__/LConn2 -- _CN_148899588_150000_CN_93173562_150000/LConn2
  _CN_148899588_150000_CN_149069221_150000/LConn3 -- T_148899588__/LConn3 -- _CN_148899588_150000_CN_93173562_150000/LConn3 -- bus102/LConn1
  _CN_148899588_150000_CN_149069221_150000/RConn1 -- T_149069221__/LConn1 -- _CN_149069221_150000_CN_148899598_150000/RConn1 -- _CN_149026599_150000_CN_149069221_150000/LConn1
  _CN_148899588_150000_CN_149069221_150000/RConn2 -- T_149069221__/LConn2 -- _CN_149069221_150000_CN_148899598_150000/RConn2 -- _CN_149026599_150000_CN_149069221_150000/LConn2
  _CN_148899588_150000_CN_149069221_150000/RConn3 -- T_149069221__/LConn3 -- _CN_149069221_150000_CN_148899598_150000/RConn3 -- bus103/LConn1 -- _CN_149026599_150000_CN_149069221_150000/LConn3
  _CN_148899588_150000_CN_93173562_150000/RConn1 -- T_93173562__/LConn1 -- _CN_93173562_150000_CN_93172457_150000/LConn1
  _CN_148899588_150000_CN_93173562_150000/RConn2 -- T_93173562__/LConn2 -- _CN_93173562_150000_CN_93172457_150000/LConn2
  _CN_148899588_150000_CN_93173562_150000/RConn3 -- T_93173562__/LConn3 -- _CN_93173562_150000_CN_93172457_150000/LConn3 -- bus104/LConn1
  _CN_129452806_150000_CN_129452815_150000/RConn1 -- T_129452815__/LConn1 -- _CN_129452812_150000_CN_129452815_150000/RConn1 -- _CN_129452815_150000_CN_149672244_150000/LConn1
  _CN_129452806_150000_CN_129452815_150000/RConn2 -- T_129452815__/LConn2 -- _CN_129452812_150000_CN_129452815_150000/RConn2 -- _CN_129452815_150000_CN_149672244_150000/LConn2
  _CN_129452806_150000_CN_129452815_150000/RConn3 -- T_129452815__/LConn3 -- _CN_129452812_150000_CN_129452815_150000/RConn3 -- _CN_129452815_150000_CN_149672244_150000/LConn3 -- bus105/LConn1
  T_148899591__/LConn1 -- _CN_148899591_150000_CN_148899598_150000/RConn1
  T_148899591__/LConn2 -- _CN_148899591_150000_CN_148899598_150000/RConn2
  _CN_148899591_150000_CN_148899598_150000/RConn3 -- T_148899591__/LConn3 -- bus106/LConn1
  T_93061385__/LConn1 -- _CN_93061385_150000_CN_93061390_150000/RConn1
  T_93061385__/LConn2 -- _CN_93061385_150000_CN_93061390_150000/RConn2
  _CN_93061385_150000_CN_93061390_150000/RConn3 -- T_93061385__/LConn3 -- bus107/LConn1
  T_115027244__/LConn1 -- _CN_93061390_150000_CN_115027244_150000/RConn1
  T_115027244__/LConn2 -- _CN_93061390_150000_CN_115027244_150000/RConn2
  _CN_93061390_150000_CN_115027244_150000/RConn3 -- T_115027244__/LConn3 -- bus108/LConn1
  _CN_129452815_150000_CN_149672244_150000/RConn1 -- T_149672244__Κέντρο_Υπερυψηλής_Τάσης_Τρικάλων/RConn1 -- _CN_149672242_150000_CN_149672244_150000/LConn1 -- L_149672244/LConn1
  _CN_129452815_150000_CN_149672244_150000/RConn2 -- T_149672244__Κέντρο_Υπερυψηλής_Τάσης_Τρικάλων/RConn2 -- _CN_149672242_150000_CN_149672244_150000/LConn2 -- L_149672244/LConn2
  _CN_129452815_150000_CN_149672244_150000/RConn3 -- T_149672244__Κέντρο_Υπερυψηλής_Τάσης_Τρικάλων/RConn3 -- _CN_149672242_150000_CN_149672244_150000/LConn3 -- L_149672244/LConn3 -- bus109/LConn1
  _CN_149026599_150000_CN_149069221_150000/RConn1 -- T_149026599__Σταθμός_Ηλεκτρικού_Ρεύματος_του_Άγρα/LConn1 -- _CN_149026599_150000_CN_171506480_150000/LConn1 -- _CN_149026599_150000_CN_149026603_150000/RConn1
  _CN_149026599_150000_CN_149069221_150000/RConn2 -- T_149026599__Σταθμός_Ηλεκτρικού_Ρεύματος_του_Άγρα/LConn2 -- _CN_149026599_150000_CN_171506480_150000/LConn2 -- _CN_149026599_150000_CN_149026603_150000/RConn2
  _CN_149026599_150000_CN_149069221_150000/RConn3 -- T_149026599__Σταθμός_Ηλεκτρικού_Ρεύματος_του_Άγρα/LConn3 -- _CN_149026599_150000_CN_171506480_150000/LConn3 -- bus110/LConn1 -- _CN_149026599_150000_CN_149026603_150000/RConn3
  _CN_149026599_150000_CN_171506480_150000/RConn1 -- T_171506480__Σταθμός_μετασχηματιστής_ρεύματος_Αμυνταίου/RConn1 -- _CN_171506480_150000_CN_93368205_150000/LConn1 -- L_171506480/LConn1 -- _CN_171506480_150000_CN_93172457_150000/LConn1
  _CN_149026599_150000_CN_171506480_150000/RConn2 -- T_171506480__Σταθμός_μετασχηματιστής_ρεύματος_Αμυνταίου/RConn2 -- _CN_171506480_150000_CN_93368205_150000/LConn2 -- L_171506480/LConn2 -- _CN_171506480_150000_CN_93172457_150000/LConn2
  _CN_149026599_150000_CN_171506480_150000/RConn3 -- T_171506480__Σταθμός_μετασχηματιστής_ρεύματος_Αμυνταίου/RConn3 -- _CN_171506480_150000_CN_93368205_150000/LConn3 -- L_171506480/LConn3 -- bus111/LConn1 -- _CN_171506480_150000_CN_93172457_150000/LConn3
  _CN_171506480_150000_CN_93172457_150000/RConn1 -- G_93172457_Ατμοηλεκτρικος_Σταθμός_Πτολεμαΐδας/RConn1 -- _CN_149481032_150000_CN_93172457_150000/RConn1 -- _CN_135177715_150000_CN_93172457_150000/RConn1 -- _CN_93173562_150000_CN_93172457_150000/RConn1
  _CN_171506480_150000_CN_93172457_150000/RConn2 -- G_93172457_Ατμοηλεκτρικος_Σταθμός_Πτολεμαΐδας/RConn2 -- _CN_149481032_150000_CN_93172457_150000/RConn2 -- _CN_135177715_150000_CN_93172457_150000/RConn2 -- _CN_93173562_150000_CN_93172457_150000/RConn2
  _CN_171506480_150000_CN_93172457_150000/RConn3 -- G_93172457_Ατμοηλεκτρικος_Σταθμός_Πτολεμαΐδας/RConn3 -- _CN_149481032_150000_CN_93172457_150000/RConn3 -- _CN_135177715_150000_CN_93172457_150000/RConn3 -- bus112/LConn1 -- _CN_93173562_150000_CN_93172457_150000/RConn3
  T_93368205__/LConn1 -- _CN_171506480_150000_CN_93368205_150000/RConn1
  T_93368205__/LConn2 -- _CN_171506480_150000_CN_93368205_150000/RConn2
  _CN_171506480_150000_CN_93368205_150000/RConn3 -- T_93368205__/LConn3 -- bus113/LConn1
  T_149672242__/LConn1 -- _CN_149672242_150000_CN_149672244_150000/RConn1
  T_149672242__/LConn2 -- _CN_149672242_150000_CN_149672244_150000/RConn2
  _CN_149672242_150000_CN_149672244_150000/RConn3 -- T_149672242__/LConn3 -- bus114/LConn1
  T_136549181__/LConn1 -- _CN_136549175_150000_CN_136549181_150000/RConn1
  T_136549181__/LConn2 -- _CN_136549175_150000_CN_136549181_150000/RConn2
  _CN_136549175_150000_CN_136549181_150000/RConn3 -- T_136549181__/LConn3 -- bus115/LConn1
  T_96759614__/LConn1 -- _CN_96759614_150000_CN_128799211_150000/RConn1
  T_96759614__/LConn2 -- _CN_96759614_150000_CN_128799211_150000/RConn2
  _CN_96759614_150000_CN_128799211_150000/RConn3 -- T_96759614__/LConn3 -- bus116/LConn1
  T_93906290__/LConn1 -- _CN_93906290_150000_CN_93906327_150000/LConn1
  T_93906290__/LConn2 -- _CN_93906290_150000_CN_93906327_150000/LConn2
  _CN_93906290_150000_CN_93906327_150000/LConn3 -- T_93906290__/LConn3 -- bus117/LConn1
  T_93906327__/LConn1 -- _CN_93906290_150000_CN_93906327_150000/RConn1
  T_93906327__/LConn2 -- _CN_93906290_150000_CN_93906327_150000/RConn2
  _CN_93906290_150000_CN_93906327_150000/RConn3 -- T_93906327__/LConn3 -- bus118/LConn1
  T_136369149__/LConn1 -- _CN_136543640_150000_CN_136369149_150000/RConn1
  T_136369149__/LConn2 -- _CN_136543640_150000_CN_136369149_150000/RConn2
  _CN_136543640_150000_CN_136369149_150000/RConn3 -- T_136369149__/LConn3 -- bus119/LConn1
  T_219975140__/LConn1 -- _CN_219975140_150000_CN_135177715_150000/RConn1
  T_219975140__/LConn2 -- _CN_219975140_150000_CN_135177715_150000/RConn2
  _CN_219975140_150000_CN_135177715_150000/RConn3 -- T_219975140__/LConn3 -- bus120/LConn1
  _CN_93383685_400000_CN_15642023_150000/RConn1 -- T_93383685__/LConn1 -- _CN_93383685_400000_CN_249066440_400000/LConn1 -- _CN_93383685_400000_CN_86577898_400000/LConn1 -- _CN_93383685_400000_CN_149672244_400000/LConn1 -- _CN_93383685_400000_CN_15641949_400000/LConn1 -- _CN_93383685_400000_CN_171506480_400000/LConn1
  _CN_93383685_400000_CN_15642023_150000/RConn2 -- T_93383685__/LConn2 -- _CN_93383685_400000_CN_249066440_400000/LConn2 -- _CN_93383685_400000_CN_86577898_400000/LConn2 -- _CN_93383685_400000_CN_149672244_400000/LConn2 -- _CN_93383685_400000_CN_15641949_400000/LConn2 -- _CN_93383685_400000_CN_171506480_400000/LConn2
  _CN_93383685_400000_CN_15642023_150000/RConn3 -- T_93383685__/LConn3 -- _CN_93383685_400000_CN_249066440_400000/LConn3 -- bus121/LConn1 -- _CN_93383685_400000_CN_86577898_400000/LConn3 -- _CN_93383685_400000_CN_149672244_400000/LConn3 -- _CN_93383685_400000_CN_15641949_400000/LConn3 -- _CN_93383685_400000_CN_171506480_400000/LConn3
  _CN_93383685_400000_CN_86577898_400000/RConn1 -- T_86577898__/LConn1 -- _CN_85526073_400000_CN_86577898_400000/LConn1 -- _CN_93119207_400000_CN_86577898_400000/LConn1
  _CN_93383685_400000_CN_86577898_400000/RConn2 -- T_86577898__/LConn2 -- _CN_85526073_400000_CN_86577898_400000/LConn2 -- _CN_93119207_400000_CN_86577898_400000/LConn2
  _CN_93383685_400000_CN_86577898_400000/RConn3 -- T_86577898__/LConn3 -- _CN_85526073_400000_CN_86577898_400000/LConn3 -- _CN_93119207_400000_CN_86577898_400000/LConn3 -- bus122/LConn1
  _CN_93383685_400000_CN_149672244_400000/RConn1 -- T_149672244__Κέντρο_Υπερυψηλής_Τάσης_Τρικάλων/LConn1 -- _CN_149672244_400000_CN_85518393_400000/LConn1 -- Γραμμή_400_kV_ΚΥΤ_Αράχθου___ΚΥΤ_Τρικάλων_CN_149672244_400000_CN_140248148_400000/LConn1
  _CN_93383685_400000_CN_149672244_400000/RConn2 -- T_149672244__Κέντρο_Υπερυψηλής_Τάσης_Τρικάλων/LConn2 -- _CN_149672244_400000_CN_85518393_400000/LConn2 -- Γραμμή_400_kV_ΚΥΤ_Αράχθου___ΚΥΤ_Τρικάλων_CN_149672244_400000_CN_140248148_400000/LConn2
